simulink model "ES241A_MotAg2Meas"  (R2013b)
settings: Solver=FixedStepDiscrete  SolverMode=SingleTasking  StartTime=0.0  StopTime=1  FixedStep=0.002  RelTol=1e-3
undefined symbols (not defined in the file): ARCHGLBPRM_2PI_ULS_F32, FLTINJ_MOTAG2MEAS_MOTAG2MECL, MOTAG2ANSINCOSFLTFAILSTEP_CNT_U16, MOTAG2ANSINCOSFLTPASSSTEP_CNT_U16, MotAg2MeasOffs, MOTAG2MECLMAX_MOTREV_F32, MOTAG2MECLMIN_MOTREV_F32, NtcNr1, NtcSts1, sigbuilder_block, VALMAXERR_VOLTSQD_F32, VALMINERR_VOLTSQD_F32
libraries: simulink x12, NxtrLim x2, FloatToFixd x1, NxtrMath x1
(part 1 of 3)
settings Model: reqMgrSettings="100 S'doors','misc'{{S'surrogatepath','savemodel','savesurrogate','updateLinks','doorsLinks2sl','slLinks2Doors','purgeDoors','purgeSimulink','detaillevel','surrogateId','synctime'{{T\"./$ModelName$\",M[1],M[1],M[0],M[0],M[0],M[0],M[0],M[1],T\"\",T\"\"}},S'mode','pathStorage'{{T\"generic\",T\"modelRelative\"}}}}"  PauseTimes=0.04  Creator=KPIT  LastModifiedBy=TZBSJD
settings SolverCC: AutoInsertRateTranBlk=on  InsertRTBMode=Always
settings DataIOCC: LimitDataPoints=off  SaveFormat=Structure  ReturnWorkspaceOutputs=on
settings OptimizationCC: BlockReduction=off  InlineParams=on  ZeroExternalMemoryAtStartup=off  ZeroInternalMemoryAtStartup=off  OptimizeModelRefInitCode=on  LifeSpan=1
settings DebuggingCC: SignalInfNanChecking=error  SignalRangeChecking=warning  UnderspecifiedInitializationDetection=Simplified  SolverPrmCheckMsg=error  InheritedTsInSrcMsg=error  DiscreteInheritContinuousMsg=error  SingleTaskRateTransMsg=error  TasksWithSamePriorityMsg=error  SigSpecEnsureSampleTimeMsg=error  CheckMatrixSingularityMsg=error  ParameterUnderflowMsg=error  ParameterPrecisionLossMsg=error  ParameterTunabilityLossMsg=error  FixptConstUnderflowMsg=warning  FixptConstOverflowMsg=warning  VectorMatrixConversionMsg=error  SignalLabelMismatchMsg=error  UnconnectedInputMsg=error  UnconnectedOutputMsg=error  UnconnectedLineMsg=error  SFcnCompatibilityMsg=error  UniqueDataStoreMsg=warning  BusObjectLabelMismatch=error  RootOutportRequireBusObject=error  AssertControl=DisableAll  ModelReferenceIOMsg=error  ModelReferenceVersionMismatchMessage=warning  ModelReferenceIOMismatchMessage=error  ModelReferenceCSMismatchMessage=warning  ModelReferenceDataLoggingMessage=error  StateNameClashWarn=warning  StrictBusMsg=ErrorOnBusTreatedAsVector  NonBusSignalsTreatedAsBus=error  SFUnexpectedBacktrackingDiag=error  SFInvalidInputDataAccessInChartInitDiag=error  SFNoUnconditionalDefaultTransitionDiag=error  SFTransitionOutsideNaturalParentDiag=error  SFUnconditionalTransitionShadowingDiag=error  SFUndirectedBroadcastEventsDiag=error
settings ModelReferenceCC: ModelReferenceNumInstancesAllowed=Single
settings SFSimCC: SimGenImportedTypeDefs=on
settings RTWCC: SystemTargetFile=autosar.tlc  GenCodeOnly=on  TemplateMakefile=ert_default_tmf  Description=AUTOSAR  GenerateReport=on  ProcessScript=autosar_make_rtw_hook  LaunchReport=on
settings CodeAppCC: GenerateComments=off  IgnoreCustomStorageClasses=off  CustomSymbolStrType=$N$R$M  CustomSymbolStrBlkIO=$N$M  SimulinkBlockComments=off
settings STFCustomTargetCC: ParMdlRefBuildCompliant=on  CompOptLevelCompliant=on  IncludeMdlTerminateFcn=off  CombineOutputUpdateFcns=on  SuppressErrorStatus=on  ERTFirstTimeCompliant=on  ERTCustomFileBanners=on  SupportNonFinite=off  SupportComplex=off  SupportContinuousTime=off  SupportNonInlinedSFcns=off  MATLABClassNameForMDSCustomization=Simulink.SoftwareTarget.ERTCustomization  AutosarCompliant=on  GRTInterface=off  SystemTargetFile=autosar.tlc
settings ERTTargetCC: CodeReplacementLibrary=ANSI_C  ConcurrentExecutionCompliant=off  IncludeMdlTerminateFcn=off  SuppressErrorStatus=on  SupportNonFinite=off  SupportComplex=off  ModelStepFunctionPrototypeControlCompliant=off  CPPClassGenCompliant=off  AutosarCompliant=on  InlinedParameterPlacement=NonHierarchical  ERTCustomFileTemplate=example_file_process.tlc  EnableUserReplacementTypes=on

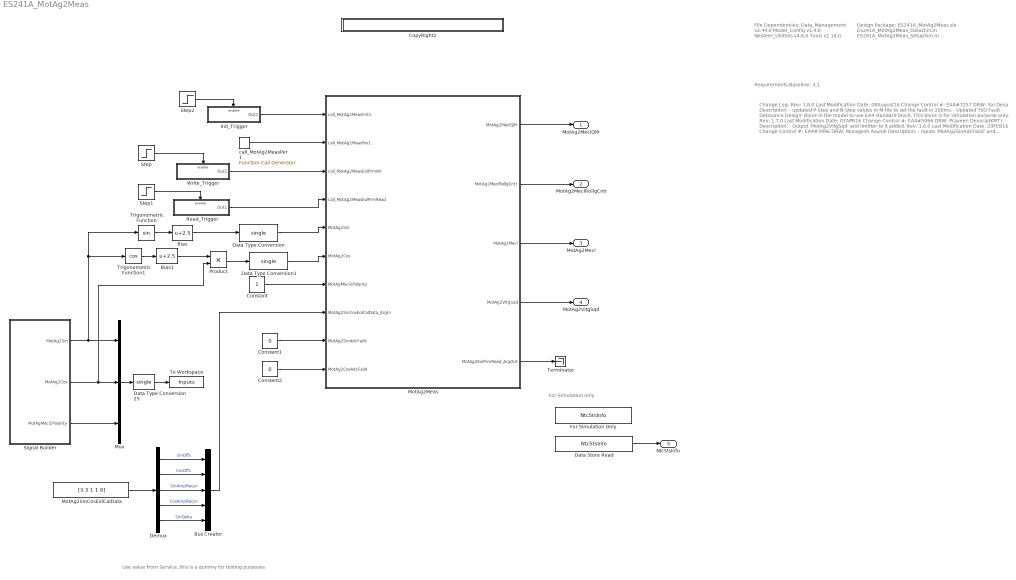
== system ES241A_MotAg2Meas ==
  note: Requirements Baseline: 3.1
  note: File Dependencies:
      |
      | Data_Management v2.44.0
      | Model_Config v1.4.0
      | Nexteer_Utilities v4.6.0
      | Tools v1.14.0
  note: Change Log:
      | Rev: 1.8.0
      | Last Modification Date: 08August16
      | Change Control #: EA4#7257
      | DRW: Sai Desu
      | Description:
      |      - updated P-Step and N-Step values in M-file to set the fault in 200ms.
      |      - Updated 'ISO Fault Debounce Design' Block in the model to use EA4 standard block.
      |        This block is for simulation purpose only.
      |
      | Rev: 1.7.0
      | Last Modification Date: 07APR16
      | Change Control #: EA4#5066
      | DRW: Praveen Devaraj(KPIT)
      | Description:
      |      - Output 'MotAg2VltgSqd' and limitter to it added.
      |
      | Rev: 1.6.0
      | Last Modification Date: 29FEB16
      | Change Control #: EA4#3996
      | DRW: Muragesh Asundi
      | Description:
      |      - Inputs 'MotAg2SinAdcFaild' and 'MotAg2CosAdcFaild' and logic related
      |        to these inputs added
      |
      | Rev: 1.5.0
      | Last Modification Date: 16DEC15
      | Change Control #: EA4#2797
      | DRW: Keyurkumar Gondaliya/Muragesh Asundi
      | Description:
      |      - Input 'MtrAg2SinCosEolCalDataCrc_ArgIn' and output 'MotAg2SinCosWrResp_ArgOut' removed
      |      - 'MtrAg2EolPrmReadCrc_ArgOut' and logic related to it removed. DD updated.
      |      - Fixed anlomaly CR EA4#2565
      |
      | Rev: 1.4.0
      | Last Modification Date: 18NOV15
      | Change Control #: EA4#2526
      | DRW: Erlenbeck
      | Description:
      | 	Change the output type of MotAg2Mecl from f32 to u0p16
      |
      | Rev: 1.3.0
      | Last Modification Date: 10.26.2015
      | Change Control #: EA4#1460
      | DRW: Muragesh Asundi
      | Description:
      | - Remove Mod block
      | - Change CRC length from 10 to 20
      | - Naming conventions for Nstep & Pstep changed as PASS and Fail step
      | - Add limitter for output 'MotAg2Mecl'
      |
      | Rev: 1.2.0
      | Last Modification Date: 08.27.2015
      | Change Control #: EA4#1421
      | DRW: Muragesh Asundi
      | Description:
      | - Changed I/O from the service functions from an array of f32 to the EOL parameter struct
      | - Removed 2 from the struct
      | - Changed IO signals names from MtrPos to MotAg
      | - PIM MotAg2MeclRollgCntrPrev added
      |
      | Rev: 1.1.0
      | Last Modification Date: 08.24.2015
      | Change Control #: EA4#1356
      | DRW: Muragesh Asundi
      | Description:
      | - Added Fault Injection block for output MotAg2Mecl
      |
      | v1.0.0
      | Date: 18-Aug-2015
      | Change Control #: EA4#1007
      | DRW:  Aditya Tikekar
      | Description:
      | - Initial Release of EA3 1.0.0
  note: Design Package:
      |
      | ES241A_MotAg2Meas.slx
      | ES241A_MotAg2Meas_DataDict.m
      | ES241A_MotAg2Meas_SetupSim.m
  note: Use value from Service, this is a dummy for testing purposes
  note: For Simulation only
  Bias : Bias  Bias=2.5
  Bias1 : Bias  Bias=2.5
  Bus Creator : BusCreator  Inputs='SinOffs','CosOffs','SinAmpRecpr','CosAmpRecpr','SinDelta'  OutDataTypeStr=Bus: MotAgMeasEolPrmRec1  NonVirtualBus=on
  Constant : Constant
  Constant1 : Constant  Value=0  OutDataTypeStr=boolean
  Constant2 : Constant  Value=0  OutDataTypeStr=boolean
  CopyRight2 : Subsystem  Description=|  mask(Copyright Information){none=on}
      | Copyright info block.                                               
      |                                                                     
      | Place copyright information at the top of every subsystem in design.
      mask prompts: none "No parameters"
      mask help: Place copyright information at the top of every subsystem in design.
      mask Display:
      | NxtrConf = 'Nexteer Confidential';
      | 
      | sys = bdroot; %handle for the current model ("system")
      | first = get_param(sys,'Created');
      | if(isempty(first))
      |     first = datestr(now,'yyyy');
      | else
      |     first = first(end-3:end);  %year is last four digits
      | end
      | 
      | last = get_param(sys,'LastModifiedDate');
      | if isempty(last)
      |     last = datestr(now,'yyyy');
      | else
      |     last = last(end-3:end);
      | end
      | 
      | if strcmp(first,last)
      |     fprintf('%s -- Copyright %s Nexteer',NxtrConf,first)
      | else
      |     fprintf('%s -- %s%s- %s Nexteer',NxtrConf,char(169),first,last)
      | end
  Data Store Read : DataStoreRead  DataStoreName=NtcStsInfo  SampleTime=0.002
  Data Type Conversion : DataTypeConversion  OutDataTypeStr=single
  Data Type Conversion1 : DataTypeConversion  OutDataTypeStr=single
  Data Type Conversion25 : DataTypeConversion  OutDataTypeStr=single
  Demux : Demux  Outputs=5
  For Simulation Only : DataStoreMemory  DataStoreName=NtcStsInfo  ReadBeforeWriteMsg=warning  WriteAfterWriteMsg=warning  WriteAfterReadMsg=warning
  Init_Trigger : Subsystem  TreatAsAtomicUnit=on
  MotAg2Meas : Subsystem
  MotAg2SinCosEolCalData : Constant  Value=[3 3 1 1 0]  OutDataTypeStr=single
  Mux : Mux  Inputs=3
  Product : Product
  Read_Trigger : Subsystem  TreatAsAtomicUnit=on
  Signal Builder : Subsystem  Tag=STV Subsys  LoadFcn=sigbuilder_block('load');  StartFcn=sigbuilder_block('start');  StopFcn=sigbuilder_block('stop');  ClipboardFcn=sigbuilder_block('clipboard');  mask(Sigbuilder block){}
      mask help: Simulink:masks:SigbuilderBlock_MD
      mask init:
      | if ~strcmp(get_param(bdroot(gcbh),'SimulationStatus'),'stopped') tuvar = sigbuilder_block('maskInit'); end
      settings: CopyFcn=sigbuilder_block('copy');  DeleteFcn=sigbuilder_block('delete');  ModelCloseFcn=sigbuilder_block('modelClose');  PreSaveFcn=sigbuilder_block('preSave');  PauseFcn=sigbuilder_block('pause');  ContinueFcn=sigbuilder_block('continue');  NameChangeFcn=sigbuilder_block('namechange');  OpenFcn=sigbuilder_block('open',[-1024.5 0 1024.5 519 ]);  CloseFcn=sigbuilder_block('close');
      mask Display: plot(0, 0, 100, 100,[2, 2, 32, 32, 2], [68, 8, 8, 68, 68],[32, 2], [38, 38], [32, 19, 2],[53, 60, 44], [32, 17, 17, 2],[16, 16, 31, 31]);txt = getActiveGroup(gcbh);text(2, 100, txt,'verticalAlignment', 'top');
  Step : Step  Time=0.25  SampleTime=0
  Step1 : Step  Time=0.006  SampleTime=0
  Step2 : Step  Time=0.002  Before=1  After=0  SampleTime=0
  Terminator : Terminator
  To Workspace : ToWorkspace  VariableName=Inputs  SampleTime=-1
  Trigonometric Function : Trigonometry
  Trigonometric Function1 : Trigonometry  Operator=cos
  Write_Trigger : Subsystem  TreatAsAtomicUnit=on
  call_MotAg2MeasPer1 : simulink/Ports & Subsystems/Function-Call Generator  RequirementInfo={} %GIDa_bc46352c_0424_4e0d_b48f_57630b448788  sample_time=0.002  numberOfIterations=1
  MotAg2MeclQlfr : Outport  RequirementInfo={} %GIDa_13339e60_d901_415b_99de_5a5f823e821e
  MotAg2MeclRollgCntr : Outport  RequirementInfo={} %GIDa_64b1d497_6b46_497b_9639_71fa2240e4cb  Port=2
  MotAg2Mecl : Outport  RequirementInfo={} %GIDa_77db205e_a8cc_41ed_9223_bd045923b052  Port=3
  MotAg2VltgSqd : Outport  Port=4
  NtcStsInfo : Outport  RequirementInfo={} %GIDa_305790cc_b4da_485d_acf3_4b5d9228ea47  Port=5
  wires:
  call_MotAg2MeasPer1/1 -> MotAg2Meas/2(call_MotAg2MeasPer1)
  MotAg2Meas/5(MotAg2EolPrmRead_ArgOut) -> Terminator/1
  Mux/1 -> Data Type Conversion25/1
  Data Type Conversion25/1 -> To Workspace/1
  Constant/1 -> MotAg2Meas/7(MotAgMecl2Polarity)
  Bias/1 -> Data Type Conversion/1
  Step/1 -> Write_Trigger/Enable
  Step1/1 -> Read_Trigger/Enable
  Write_Trigger/1(Out1) -> MotAg2Meas/3(call_MotAg2MeasEolPrmWr)
  Read_Trigger/1(Out1) -> MotAg2Meas/4(call_MotAg2MeasEolPrmRead)
  Step2/1 -> Init_Trigger/Enable
  Init_Trigger/1(Out1) -> MotAg2Meas/1(call_MotAg2MeasInit1)
  Signal Builder/1(MotAg2Sin) -> Mux/1, Trigonometric Function/1, Trigonometric Function1/1
  Signal Builder/3(MotAgMecl2Polarity) -> Mux/3
  Signal Builder/2(MotAg2Cos) -> Product/2, Mux/2
  MotAg2Meas/1(MotAg2MeclQlfr) -> MotAg2MeclQlfr/1
  MotAg2Meas/2(MotAg2MeclRollgCntr) -> MotAg2MeclRollgCntr/1
  MotAg2Meas/3(MotAg2Mecl) -> MotAg2Mecl/1
  Trigonometric Function/1 -> Bias/1
  Trigonometric Function1/1 -> Bias1/1
  Bias1/1 -> Product/1
  Data Type Conversion/1 -> MotAg2Meas/5(MotAg2Sin)
  Data Type Conversion1/1 -> MotAg2Meas/6(MotAg2Cos)
  Product/1 -> Data Type Conversion1/1
  Demux/5 -> Bus Creator/5  "SinDelta"
  Demux/4 -> Bus Creator/4  "CosAmpRecpr"
  Demux/2 -> Bus Creator/2  "CosOffs"
  Demux/3 -> Bus Creator/3  "SinAmpRecpr"
  Demux/1 -> Bus Creator/1  "SinOffs"
  MotAg2SinCosEolCalData/1 -> Demux/1
  Bus Creator/1 -> MotAg2Meas/8(MotAg2SinCosEolCalData_ArgIn)
  Constant2/1 -> MotAg2Meas/10(MotAg2CosAdcFaild)
  Constant1/1 -> MotAg2Meas/9(MotAg2SinAdcFaild)
  Data Store Read/1 -> NtcStsInfo/1
  MotAg2Meas/4(MotAg2VltgSqd) -> MotAg2VltgSqd/1

== system ES241A_MotAg2Meas/CopyRight2 ==

== system ES241A_MotAg2Meas/Init_Trigger ==
  Enable : EnablePort
  Function-Call Generator1 : simulink/Ports & Subsystems/Function-Call Generator  sample_time=0  numberOfIterations=1
  Out1 : Outport
  wires:
  Function-Call Generator1/1 -> Out1/1

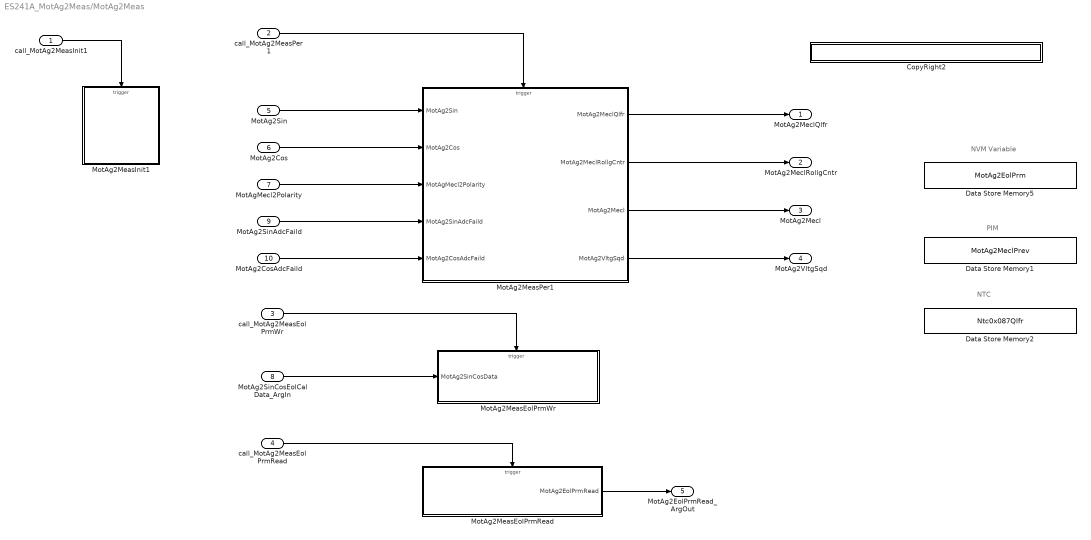
== system ES241A_MotAg2Meas/MotAg2Meas ==
  note: PIM
  note: NTC
  note: NVM Variable
  call_MotAg2MeasInit1 : Inport
  call_MotAg2MeasPer1 : Inport  Port=2
  call_MotAg2MeasEolPrmWr : Inport  Port=3
  call_MotAg2MeasEolPrmRead : Inport  Port=4
  MotAg2Sin : Inport  RequirementInfo={'linktype_rmi_doors' '0000cf65 (/E-STEER Core/SubSystem Specifications/Electrical Actuator/Control Module/FDD Module Requirements/EA4/ES241A_MotAg2Meas)' '#ES241A_49' 'true' 'REQ: ES241A_49' '' } %GIDa_7d298e34_c05b_439c_ad49_94e8d3b397f3  Port=5
  MotAg2Cos : Inport  RequirementInfo={'linktype_rmi_doors' '0000cf65 (/E-STEER Core/SubSystem Specifications/Electrical Actuator/Control Module/FDD Module Requirements/EA4/ES241A_MotAg2Meas)' '#ES241A_48' 'true' 'REQ: ES241A_48' '' } %GIDa_73391b37_a5e9_4145_aca0_ac09474f9974  Port=6
  MotAgMecl2Polarity : Inport  RequirementInfo={'linktype_rmi_doors' '0000cf65 (/E-STEER Core/SubSystem Specifications/Electrical Actuator/Control Module/FDD Module Requirements/EA4/ES241A_MotAg2Meas)' '#ES241A_65' 'true' 'REQ: ES241A_65' '' } %GIDa_856eeb3a_bbb6_4880_ab78_80a15c90fc09  Port=7
  MotAg2SinCosEolCalData_ArgIn : Inport  Port=8  OutDataTypeStr=Bus: MotAgMeasEolPrmRec1
  MotAg2SinAdcFaild : Inport  RequirementInfo={'linktype_rmi_doors' '0000cf65 (/E-STEER Core/SubSystem Specifications/Electrical Actuator/Control Module/FDD Module Requirements/EA4/ES241A_MotAg2Meas)' '#ES241A_146' 'true' 'REQ: ES241A_146' '' } %GIDa_82f7f128_b8c8_49c8_b664_98de2aa09858  Port=9
  MotAg2CosAdcFaild : Inport  RequirementInfo={'linktype_rmi_doors' '0000cf65 (/E-STEER Core/SubSystem Specifications/Electrical Actuator/Control Module/FDD Module Requirements/EA4/ES241A_MotAg2Meas)' '#ES241A_145' 'true' 'REQ: ES241A_145' '' } %GIDa_a44d5a9e_6b3c_447d_b1ad_61e623b783fe  Port=10
  CopyRight2 : Subsystem  Description=|  mask(Copyright Information){none=on}
      | Copyright info block.                                               
      |                                                                     
      | Place copyright information at the top of every subsystem in design.
      mask prompts: none "No parameters"
      mask help: Place copyright information at the top of every subsystem in design.
      mask Display:
      | NxtrConf = 'Nexteer Confidential';
      | 
      | sys = bdroot; %handle for the current model ("system")
      | first = get_param(sys,'Created');
      | if(isempty(first))
      |     first = datestr(now,'yyyy');
      | else
      |     first = first(end-3:end);  %year is last four digits
      | end
      | 
      | last = get_param(sys,'LastModifiedDate');
      | if isempty(last)
      |     last = datestr(now,'yyyy');
      | else
      |     last = last(end-3:end);
      | end
      | 
      | if strcmp(first,last)
      |     fprintf('%s -- Copyright %s Nexteer',NxtrConf,first)
      | else
      |     fprintf('%s -- %s%s- %s Nexteer',NxtrConf,char(169),first,last)
      | end
  Data Store Memory1 : DataStoreMemory  DataStoreName=MotAg2MeclPrev  StateMustResolveToSignalObject=on
  Data Store Memory2 : DataStoreMemory  DataStoreName=Ntc0x087Qlfr
  Data Store Memory5 : DataStoreMemory  DataStoreName=MotAg2EolPrm  InitialValue=[]  OutDataTypeStr=Bus: MotAgMeasEolPrmRec1  StateMustResolveToSignalObject=on
  MotAg2MeasEolPrmRead : Subsystem  RequirementInfo={'linktype_rmi_doors' '0000cf65 (/E-STEER Core/SubSystem Specifications/Electrical Actuator/Control Module/FDD Module Requirements/EA4/ES241A_MotAg2Meas)' '#ES241A_135' 'true' 'REQ: ES241A_135' '' } %GIDa_cb0be6f7_2f31_479b_8294_40ee3e4aca08  TreatAsAtomicUnit=on
  MotAg2MeasEolPrmWr : Subsystem  RequirementInfo={'linktype_rmi_doors' '0000cf65 (/E-STEER Core/SubSystem Specifications/Electrical Actuator/Control Module/FDD Module Requirements/EA4/ES241A_MotAg2Meas)' '#ES241A_32' 'true' 'REQ: ES241A_32' '' } %GIDa_9fac367d_a0e4_41dd_ba23_6b4ec78d47c5
  MotAg2MeasInit1 : Subsystem  TreatAsAtomicUnit=on
  MotAg2MeasPer1 : Subsystem  ClipboardFcn=Priority=%<Priority>  TreatAsAtomicUnit=on
  MotAg2MeclQlfr : Outport  RequirementInfo={'linktype_rmi_doors' '0000cf65 (/E-STEER Core/SubSystem Specifications/Electrical Actuator/Control Module/FDD Module Requirements/EA4/ES241A_MotAg2Meas)' '#ES241A_113' 'true' 'REQ: ES241A_113' '' } %GIDa_ad4892e3_f342_4a8c_9fb3_dbca1d6629f8
  MotAg2MeclRollgCntr : Outport  RequirementInfo={'linktype_rmi_doors' '0000cf65 (/E-STEER Core/SubSystem Specifications/Electrical Actuator/Control Module/FDD Module Requirements/EA4/ES241A_MotAg2Meas)' '#ES241A_114' 'true' 'REQ: ES241A_114' '' } %GIDa_5e51ab32_dc6c_4788_a108_d1ac524f47aa  Port=2
  MotAg2Mecl : Outport  RequirementInfo={'linktype_rmi_doors' '0000cf65 (/E-STEER Core/SubSystem Specifications/Electrical Actuator/Control Module/FDD Module Requirements/EA4/ES241A_MotAg2Meas)' '#ES241A_51' 'true' 'REQ: ES241A_51' '' } %GIDa_b54aa487_7774_4247_9155_2f93ac20eae7  Port=3
  MotAg2VltgSqd : Outport  RequirementInfo={'linktype_rmi_doors' '0000cf65 (/E-STEER Core/SubSystem Specifications/Electrical Actuator/Control Module/FDD Module Requirements/EA4/ES241A_MotAg2Meas)' '#ES241A_151' 'true' 'REQ: ES241A_151' '' } %GIDa_822906ad_a1cb_4535_b465_c74a6fe6a8d1  Port=4
  MotAg2EolPrmRead_ArgOut : Outport  Port=5  OutDataTypeStr=Bus: MotAgMeasEolPrmRec1
  wires:
  call_MotAg2MeasPer1/1 -> MotAg2MeasPer1/Trigger
  MotAg2Sin/1 -> MotAg2MeasPer1/1(MotAg2Sin)
  MotAgMecl2Polarity/1 -> MotAg2MeasPer1/3(MotAgMecl2Polarity)
  MotAg2Cos/1 -> MotAg2MeasPer1/2(MotAg2Cos)
  MotAg2MeasPer1/1(MotAg2MeclQlfr) -> MotAg2MeclQlfr/1
  MotAg2MeasPer1/2(MotAg2MeclRollgCntr) -> MotAg2MeclRollgCntr/1
  MotAg2MeasPer1/3(MotAg2Mecl) -> MotAg2Mecl/1
  call_MotAg2MeasInit1/1 -> MotAg2MeasInit1/Trigger
  call_MotAg2MeasEolPrmWr/1 -> MotAg2MeasEolPrmWr/Trigger
  MotAg2MeasEolPrmRead/1(MotAg2EolPrmRead) -> MotAg2EolPrmRead_ArgOut/1
  call_MotAg2MeasEolPrmRead/1 -> MotAg2MeasEolPrmRead/Trigger
  MotAg2SinCosEolCalData_ArgIn/1 -> MotAg2MeasEolPrmWr/1(MotAg2SinCosData)
  MotAg2SinAdcFaild/1 -> MotAg2MeasPer1/4(MotAg2SinAdcFaild)
  MotAg2CosAdcFaild/1 -> MotAg2MeasPer1/5(MotAg2CosAdcFaild)
  MotAg2MeasPer1/4(MotAg2VltgSqd) -> MotAg2VltgSqd/1

== system ES241A_MotAg2Meas/Read_Trigger ==
  Enable : EnablePort
  Function-Call Generator1 : simulink/Ports & Subsystems/Function-Call Generator  sample_time=0.002  numberOfIterations=1
  Out1 : Outport
  wires:
  Function-Call Generator1/1 -> Out1/1

== system ES241A_MotAg2Meas/Signal Builder ==
  Demux : Demux  Tag=STV Demux  Outputs=3
  FromWs : FromWorkspace  Tag=STV FromWs  VariableName=tuvar  SampleTime=0
      SigBuilderData=|
      | common.afterFinalStr = 'Extrapolate'
      | common.sampleTime = 0
      | dataSet(1).timeRange = [0 1]
      | dataSet(1).name = 'MotAg2CosCmp_Calc'
      | dataSet(2).timeRange = [0 1]
      | dataSet(2).name = 'MotAg2SinCmp_Calc'
      | dataSet(3).timeRange = [0 0.04]
      | dataSet(3).name = 'CosTheta_Calc'
      | dataSet(4).timeRange = [0 0.04]
      | dataSet(4).name = 'MotAg2Mecl_Calc_Polarity_1'
      | dataSet(5).timeRange = [0 0.04]
      | dataSet(5).name = 'MotAg2Mecl_Calc_Polarity_-1'
      | dataSet(6).timeRange = [0 0.25]
      | dataSet(6).name = 'ISO_Fault'
      | dataSet(7).timeRange = [0 1]
      | dataSet(7).name = 'RollCntr>255'
      | dataSet(8).timeRange = [0 1]
      | dataSet(8).name = 'NoFault'
      | sbobj.Name = 'Signal Builder'
      | sbobj.Groups(1).Name = 'MotAg2CosCmp_Calc'
      | sbobj.Groups(1).Signals(1).Name = 'MotAg2Sin'
      | sbobj.Groups(1).Signals(1).XData = [0 0.002 0.004 0.006 0.008 0.01 0.012 0.014 0.016 0.018 0.02 0.02 0.022 0.022 0.024 0.026 0.028 0.03 0.032 0.034 0.036 0.038 0.04 0.04 1]
      | sbobj.Groups(1).Signals(1).YData = [0 2.5 4.5 5 4.5 2.5 0 2.5 4.5 5 4.5 4.45 2.3 2.5 0 2.5 4.5 5 4.5 2.5 0 2.5 4.5 1.95 1.95]
      | sbobj.Groups(1).Signals(2).Name = 'MotAg2Cos'
      | sbobj.Groups(1).Signals(2).XData = [0 0.002 0.004 0.006 0.008 0.01 0.012 0.014 0.016 0.018 0.02 0.022 0.024 0.026 0.028 0.03 0.032 0.034 0.036 0.038 0.04 1]
      | sbobj.Groups(1).Signals(2).YData = [5 4.5 2.5 0 2.5 4.5 5 4.5 2.5 0 2.5 4.5 5 4.5 2.5 0 2.5 4.5 5 4.5 2.5 2.5]
      | sbobj.Groups(1).Signals(3).Name = 'MotAgMecl2Polarity'
      | sbobj.Groups(1).Signals(3).XData = [0 0.002 0.004 0.006 0.008 0.01 0.012 0.014 0.016 0.018 0.02 0.022 0.024 0.026 0.028 0.03 0.032 0.034 0.036 0.038 0.04 1]
      | sbobj.Groups(1).Signals(3).YData = [-1 1 -1 1 -1 1 -1 0 0 0 1 -1 1 0 -1 1 -1 1 0 0 1 1]
      | sbobj.Groups(1).TimeRange = [0 1]
      | sbobj.Groups(2).Name = 'MotAg2SinCmp_Calc'
      | sbobj.Groups(2).Signals(1).Name = 'MotAg2Sin'
      | sbobj.Groups(2).Signals(1).XData = [0 0.5 0.5 1]
      | sbobj.Groups(2).Signals(1).YData = [0 6.28318 0 6.28318]
      | sbobj.Groups(2).Signals(2).Name = 'MotAg2Cos'
      | sbobj.Groups(2).Signals(2).XData = [0 0.5 0.5 1]
      | sbobj.Groups(2).Signals(2).YData = [1 1 0 0]
      | sbobj.Groups(2).Signals(3).Name = 'MotAgMecl2Polarity'
      | sbobj.Groups(2).Signals(3).XData = [0 0.002 0.004 0.006 0.008 0.01 0.012 0.014 0.016 0.018 0.02 0.022 0.024 0.026 0.028 0.03 0.032 0.034 0.036 0.038 0.04 1]
      | sbobj.Groups(2).Signals(3).YData = [-1 1 -1 1 -1 1 -1 0 0 0 1 -1 1 0 -1 1 -1 1 0 0 1 1]
      | sbobj.Groups(2).TimeRange = [0 1]
      | sbobj.Groups(3).Name = 'CosTheta_Calc'
      | sbobj.Groups(3).Signals(1).Name = 'MotAg2Sin'
      | sbobj.Groups(3).Signals(1).XData = [0 0.002 0.004 0.006 0.008 0.01 0.012 0.014 0.016 0.018 0.02 0.022 0.024 0.026 0.028 0.03 0.032 0.034 0.036 0.038 0.04]
      | sbobj.Groups(3).Signals(1).YData = [0 2.5 4.5 5 4.5 2.5 0 2.5 4.5 5 4.5 2.5 0 2.5 4.5 5 4.5 2.5 0 2.5 4.5]
      | sbobj.Groups(3).Signals(2).Name = 'MotAg2Cos'
      | sbobj.Groups(3).Signals(2).XData = [0 0.002 0.004 0.006 0.008 0.01 0.012 0.014 0.016 0.018 0.02 0.022 0.024 0.026 0.028 0.03 0.032 0.034 0.036 0.038 0.04]
      | sbobj.Groups(3).Signals(2).YData = [5 4.5 2.5 0 2.5 4.5 5 4.5 2.5 0 2.5 4.5 5 4.5 2.5 0 2.5 4.5 5 4.5 2.5]
      | sbobj.Groups(3).Signals(3).Name = 'MotAgMecl2Polarity'
      | sbobj.Groups(3).Signals(3).XData = [0 0.002 0.004 0.006 0.008 0.01 0.012 0.014 0.016 0.018 0.02 0.022 0.024 0.026 0.028 0.03 0.032 0.034 0.036 0.038 0.04]
      | sbobj.Groups(3).Signals(3).YData = [-1 1 -1 1 -1 1 -1 0 0 0 1 -1 1 0 -1 1 -1 1 0 0 1]
      | sbobj.Groups(3).TimeRange = [0 0.04]
      | sbobj.Groups(4).Name = 'MotAg2Mecl_Calc_Polarity_1'
      | sbobj.Groups(4).Signals(1).Name = 'MotAg2Sin'
      | sbobj.Groups(4).Signals(1).XData = [0 0.002 0.004 0.006 0.008 0.01 0.012 0.014 0.016 0.018 0.02 0.022 0.024 0.026 0.028 0.03 0.032 0.034 0.036 0.038 0.04]
      | sbobj.Groups(4).Signals(1).YData = [0 2.5 4.5 5 4.5 2.5 0 2.5 4.5 5 4.5 2.5 0 2.5 4.5 5 4.5 2.5 0 2.5 4.5]
      | sbobj.Groups(4).Signals(2).Name = 'MotAg2Cos'
      | sbobj.Groups(4).Signals(2).XData = [0 0.002 0.004 0.006 0.008 0.01 0.012 0.014 0.016 0.018 0.02 0.022 0.024 0.026 0.028 0.03 0.032 0.034 0.036 0.038 0.04]
      | sbobj.Groups(4).Signals(2).YData = [5 4.5 2.5 0 2.5 4.5 5 4.5 2.5 0 2.5 4.5 5 4.5 2.5 0 2.5 4.5 5 4.5 2.5]
      | sbobj.Groups(4).Signals(3).Name = 'MotAgMecl2Polarity'
      | sbobj.Groups(4).Signals(3).XData = [0 0.002 0.004 0.006 0.008 0.01 0.012 0.014 0.016 0.018 0.02 0.022 0.024 0.026 0.028 0.03 0.032 0.034 0.036 0.038 0.04]
      | sbobj.Groups(4).Signals(3).YData = [1 1 1 1 1 1 1 1 1 1 1 1 1 1 1 1 1 1 1 1 1]
      | sbobj.Groups(4).TimeRange = [0 0.04]
      | sbobj.Groups(5).Name = 'MotAg2Mecl_Calc_Polarity_-1'
      | sbobj.Groups(5).Signals(1).Name = 'MotAg2Sin'
      | sbobj.Groups(5).Signals(1).XData = [0 0.002 0.004 0.006 0.008 0.01 0.012 0.014 0.016 0.018 0.02 0.022 0.024 0.026 0.028 0.03 0.032 0.034 0.036 0.038 0.04]
      | sbobj.Groups(5).Signals(1).YData = [0 2.5 4.5 5 4.5 2.5 0 2.5 4.5 5 4.5 2.5 0 2.5 4.5 5 4.5 2.5 0 2.5 4.5]
      | sbobj.Groups(5).Signals(2).Name = 'MotAg2Cos'
      | sbobj.Groups(5).Signals(2).XData = [0 0.002 0.004 0.006 0.008 0.01 0.012 0.014 0.016 0.018 0.02 0.022 0.024 0.026 0.028 0.03 0.032 0.034 0.036 0.038 0.04]
      | sbobj.Groups(5).Signals(2).YData = [5 4.5 2.5 0 2.5 4.5 5 4.5 2.5 0 2.5 4.5 5 4.5 2.5 0 2.5 4.5 5 4.5 2.5]
      | sbobj.Groups(5).Signals(3).Name = 'MotAgMecl2Polarity'
      | sbobj.Groups(5).Signals(3).XData = [0 0.002 0.004 0.006 0.008 0.01 0.012 0.014 0.016 0.018 0.02 0.022 0.024 0.026 0.028 0.03 0.032 0.034 0.036 0.038 0.04]
      | sbobj.Groups(5).Signals(3).YData = [-1 -1 -1 -1 -1 -1 -1 -1 -1 -1 -1 -1 -1 -1 -1 -1 -1 -1 -1 -1 -1]
      | sbobj.Groups(5).TimeRange = [0 0.04]
      | sbobj.Groups(6).Name = 'ISO_Fault'
      | sbobj.Groups(6).Signals(1).Name = 'MotAg2Sin'
      | sbobj.Groups(6).Signals(1).XData = [0 0.002 0.004 0.006 0.008 0.01 0.012 0.014 0.016 0.018 0.02 0.022 0.024 0.026 0.028 0.03 0.032 0.034 0.036 0.038 0.04 0.042 0.044 0.046 0.048 0.05 0.052 0.054 0.056 0.058 0.06 0.062 0.064 0.066 0.068 0.07 0.072 0.074 0.076 0.078 0.08 0.082 0.084 0.086 0.088 0.09 0.092 0.094 0.096 0.098 0.1 0.102 0.104 0.106 0.108 0.11 0.112 0.114 0.116 0.118 0.12 0.122 0.124 0.126 0.128 0.13 0.132 0.134 0.136 0.138 0.14 0.142 0.144 0.146 0.148 0.15 0.152 0.154 0.156 0.158 0.16 0.162 0.164 0.166 0.168 0.17 0.172 0.174 0.176 0.178 0.18 0.182 0.184 0.186 0.188 0.19 0.192 0.194 0.196 0.198 0.2 0.202 0.204 0.206 0.208 0.21 0.212 0.214 0.216 0.218 0.22 0.222 0.224 0.226 0.228 0.23 0.232 0.234 0.236 0.238 0.24 0.242 0.244 0.246 0.248 0.25]
      | sbobj.Groups(6).Signals(1).YData = [0 2.5 4.5 5 4.5 2.5 0 2.5 4.5 5 4.5 2.5 0 2.5 4.5 5 4.5 2.5 0 2.5 4.5 5 4.5 2.5 0 2.5 4.5 5 4.5 2.5 0 2.5 4.5 5 4.5 2.5 0 2.5 4.5 5 4.5 2.5 0 2.5 4.5 5 4.5 2.5 0 2.5 4.5 5 4.5 2.5 0 2.5 4.5 5 4.5 2.5 0 2.5 4.5 5 4.5 2.5 0 2.5 4.5 5 4.5 2.5 0 2.5 4.5 5 4.5 2.5 0 2.5 4.5 5 4.5 2.5 0 2.5 4.5 5 4.5 2.5 0 2.5 4.5 5 4.5 2.5 0 2.5 4.5 5 4.5 2.5 0 2.5 4.5 5 4.5 2.5 0 2.5 4.5 5 4.5 2.5 0 2.5 4.5 5 4.5 2.5 0 2.5 4.5 5 4.5 2.5]
      | sbobj.Groups(6).Signals(2).Name = 'MotAg2Cos'
      | sbobj.Groups(6).Signals(2).XData = [0 0.002 0.004 0.006 0.008 0.01 0.012 0.014 0.016 0.018 0.02 0.022 0.024 0.026 0.028 0.03 0.032 0.034 0.036 0.038 0.04 0.042 0.044 0.046 0.048 0.05 0.052 0.054 0.056 0.058 0.06 0.062 0.064 0.066 0.068 0.07 0.072 0.074 0.076 0.078 0.08 0.082 0.084 0.086 0.088 0.09 0.092 0.094 0.096 0.098 0.1 0.102 0.104 0.106 0.108 0.11 0.112 0.114 0.116 0.118 0.12 0.122 0.124 0.126 0.128 0.13 0.132 0.134 0.136 0.138 0.14 0.142 0.144 0.146 0.148 0.15 0.152 0.154 0.156 0.158 0.16 0.162 0.164 0.166 0.168 0.17 0.172 0.174 0.176 0.178 0.18 0.182 0.184 0.186 0.188 0.19 0.192 0.194 0.196 0.198 0.2 0.202 0.204 0.206 0.208 0.21 0.212 0.214 0.216 0.218 0.22 0.222 0.224 0.226 0.228 0.23 0.232 0.234 0.236 0.238 0.24 0.242 0.244 0.246 0.248 0.25]
      | sbobj.Groups(6).Signals(2).YData = [5 4.5 2.5 0 2.5 4.5 5 4.5 2.5 0 2.5 4.5 5 4.5 2.5 0 2.5 4.5 5 4.5 2.5 0 2.5 4.5 5 4.5 2.5 0 2.5 4.5 5 4.5 2.5 0 2.5 4.5 5 4.5 2.5 0 2.5 4.5 5 4.5 2.5 0 2.5 4.5 5 4.5 2.5 0 2.5 4.5 5 4.5 2.5 0 2.5 4.5 5 4.5 2.5 0 2.5 4.5 5 4.5 2.5 0 2.5 4.5 5 4.5 2.5 0 2.5 4.5 5 4.5 2.5 0 2.5 4.5 5 4.5 2.5 0 2.5 4.5 5 4.5 2.5 0 2.5 4.5 5 4.5 2.5 0 2.5 4.5 5 4.5 2.5 0 2.5 4.5 5 4.5 2.5 0 2.5 4.5 5 4.5 2.5 0 2.5 4.5 5 4.5 2.5 0 2.5 4.5]
      | sbobj.Groups(6).Signals(3).Name = 'MotAgMecl2Polarity'
      | sbobj.Groups(6).Signals(3).XData = [0 0.002 0.004 0.006 0.008 0.01 0.012 0.014 0.016 0.018 0.02 0.022 0.024 0.026 0.028 0.03 0.032 0.034 0.036 0.038 0.04 0.042 0.044 0.046 0.048 0.05 0.052 0.054 0.056 0.058 0.06 0.062 0.064 0.066 0.068 0.07 0.072 0.074 0.076 0.078 0.08 0.082 0.084 0.086 0.088 0.09 0.092 0.094 0.096 0.098 0.1 0.102 0.104 0.106 0.108 0.11 0.112 0.114 0.116 0.118 0.12 0.122 0.124 0.126 0.128 0.13 0.132 0.134 0.136 0.138 0.14 0.142 0.144 0.146 0.148 0.15 0.152 0.154 0.156 0.158 0.16 0.162 0.164 0.166 0.168 0.17 0.172 0.174 0.176 0.178 0.18 0.182 0.184 0.186 0.188 0.19 0.192 0.194 0.196 0.198 0.2 0.202 0.204 0.206 0.208 0.21 0.212 0.214 0.216 0.218 0.22 0.222 0.224 0.226 0.228 0.23 0.232 0.234 0.236 0.238 0.24 0.242 0.244 0.246 0.248 0.25]
      | sbobj.Groups(6).Signals(3).YData = [-1 1 -1 1 -1 1 -1 0 0 0 1 -1 1 0 -1 1 -1 1 0 0 1 -1 1 -1 1 -1 1 -1 0 0 0 1 -1 1 0 -1 1 -1 1 0 0 1 -1 1 -1 1 -1 1 -1 0 0 0 1 -1 1 0 -1 1 -1 1 0 0 1 -1 1 -1 1 -1 1 -1 0 0 0 1 -1 1 0 -1 1 -1 1 0 0 1 -1 1 -1 1 -1 1 -1 0 0 0 1 -1 1 0 -1 1 -1 1 0 0 1 -1 1 -1 1 -1 1 -1 0 0 0 1 -1 1 0 -1 1 -1 1 0 0 1]
      | sbobj.Groups(6).TimeRange = [0 0.25]
      | sbobj.Groups(7).Name = 'RollCntr>255'
      | sbobj.Groups(7).Signals(1).Name = 'MotAg2Sin'
      | sbobj.Groups(7).Signals(1).XData = [0 0.002 0.004 0.006 0.008 0.01 0.012 0.014 0.016 0.018 0.02 0.022 ... (501 elements, 1x501)]
      | sbobj.Groups(7).Signals(1).YData = [0 2.5 4.5 5 4.5 2.5 0 2.5 4.5 5 4.5 2.5 0 2.5 4.5 5 4.5 2.5 0 2.5 4.5 5 4.5 2.5 0 2.5 4.5 5 4.5 2.5 0 2.5 4.5 5 4.5 2.5 0 2.5 4.5 5 4.5 2.5 0 2.5 4.5 5 4.5 2.5 0 2.5 4.5 5 4.5 2.5 0 2.5 4.5 5 4.5 2.5 0 2.5 4.5 5 4.5 2.5 0 2.5 4.5 5 4.5 2.5 0 2.5 4.5 5 4.5 2.5 0 2.5 4.5 5 4.5 2.5 0 2.5 4.5 5 4.5 2.5 0 2.5 4.5 5 4.5 2.5 0 2.5 4.5 5 4.5 2.5 0 2.5 4.5 5 4.5 2.5 0 2.5 4.5 5 4.5 2.5 0 2.5 4.5 5 4.5 2.5 0 2.5 4.5 5 4.5 2.5 0 2.5 4.5 5 4.5 2.5 0 2.5 4.5 5 4.5 2.5 0 2.5 4.5 5 4.5 2.5 0 2.5 4.5 5 4.5 2.5 0 2.5 4.5 5 4.5 2.5 0 2.5 4.5 5 4.5 2.5 0 2.5 4.5 5 4.5 2.5 0 2.5 4.5 5 4.5 2.5 0 2.5 4.5 5 4.5 2.5 0 2.5 4.5 5 4.5 2.5 0 2.5 4.5 5 4.5 2.5 0 2.5 4.5 5 4.5 2.5 0 2.5 4.5 5 4.5 2.5 0 2.5 4.5 5 4.5 2.5 0 2.5 4.5 5 4.5 2.5 0 2.5 4.5 5 4.5 2.5 0 2.5 4.5 5 4.5 2.5 0 2.5 4.5 5 4.5 2.5 0 2.5 4.5 5 4.5 2.5 0 2.5 4.5 5 4.5 2.5 0 2.5 4.5 5 4.5 2.5 0 2.5 4.5 5 4.5 2.5 0 2.5 4.5 5 4.5 2.5 0 2.5 4.5 5 4.5 2.5 0 2.5 4.5 5 4.5 2.5 0 2.5 4.5 5 4.5 2.5 0 2.5 4.5 5 4.5 2.5 0 2.5 4.5 5 4.5 2.5 0 2.5 4.5 5 4.5 2.5 0 2.5 4.5 5 4.5 2.5 0 2.5 4.5 5 4.5 2.5 0 2.5 4.5 5 4.5 2.5 0 2.5 4.5 5 4.5 2.5 0 2.5 4.5 5 4.5 2.5 0 2.5 4.5 5 4.5 2.5 0 2.5 4.5 5 4.5 2.5 0 2.5 4.5 5 4.5 2.5 0 2.5 4.5 5 4.5 2.5 0 2.5 4.5 5 4.5 2.5 0 2.5 4.5 5 4.5 2.5 0 2.5 4.5 5 4.5 2.5 0 2.5 4.5 5 0 2.5 4.5 5 4.5 2.5 0 2.5 4.5 5 4.5 2.5 0 2.5 4.5 5 4.5 2.5 0 2.5 4.5 5 4.5 2.5 0 2.5 4.5 5 4.5 2.5 0 2.5 4.5 5 4.5 2.5 0 2.5 4.5 5 4.5 2.5 0 2.5 4.5 5 4.5 2.5 0 2.5 4.5 5 4.5 2.5 0 2.5 4.5 5 4.5 2.5 0 2.5 4.5 5 4.5 2.5 0 2.5 4.5 5 4.5 2.5 0 2.5 4.5 5 4.5 2.5 0 2.5 4.5 5 4.5 2.5 0 2.5 4.5 5 4.5 2.5 0 2.5 4.5 5 4.5 2.5 0 2.5 4.5 5 4.5 2.5 0 2.5 4.5 5 4.5 2.5 0 2.5 4.5 5 4.5 2.5 0 2.5 4.5 5 4.5 2.5 0 2.5 4.5 5 4.5]
      | sbobj.Groups(7).Signals(2).Name = 'MotAg2Cos'
      | sbobj.Groups(7).Signals(2).XData = [0 0.002 0.004 0.006 0.008 0.01 0.012 0.014 0.016 0.018 0.02 0.022 ... (501 elements, 1x501)]
      | sbobj.Groups(7).Signals(2).YData = [5 4.5 2.5 0 2.5 4.5 5 4.5 2.5 0 2.5 4.5 5 4.5 2.5 0 2.5 4.5 5 4.5 2.5 0 2.5 4.5 5 4.5 2.5 0 2.5 4.5 5 4.5 2.5 0 2.5 4.5 5 4.5 2.5 0 2.5 4.5 5 4.5 2.5 0 2.5 4.5 5 4.5 2.5 0 2.5 4.5 5 4.5 2.5 0 2.5 4.5 5 4.5 2.5 0 2.5 4.5 5 4.5 2.5 0 2.5 4.5 5 4.5 2.5 0 2.5 4.5 5 4.5 2.5 0 2.5 4.5 5 4.5 2.5 0 2.5 4.5 5 4.5 2.5 0 2.5 4.5 5 4.5 2.5 0 2.5 4.5 5 4.5 2.5 0 2.5 4.5 5 4.5 2.5 0 2.5 4.5 5 4.5 2.5 0 2.5 4.5 5 4.5 2.5 0 2.5 4.5 5 4.5 2.5 0 2.5 4.5 5 4.5 2.5 0 2.5 4.5 5 4.5 2.5 0 2.5 4.5 5 4.5 2.5 0 2.5 4.5 5 4.5 2.5 0 2.5 4.5 5 4.5 2.5 0 2.5 4.5 5 4.5 2.5 0 2.5 4.5 5 4.5 2.5 0 2.5 4.5 5 4.5 2.5 0 2.5 4.5 5 4.5 2.5 0 2.5 4.5 5 4.5 2.5 0 2.5 4.5 5 4.5 2.5 0 2.5 4.5 5 4.5 2.5 0 2.5 4.5 5 4.5 2.5 0 2.5 4.5 5 4.5 2.5 0 2.5 4.5 5 4.5 2.5 0 2.5 4.5 5 4.5 2.5 0 2.5 4.5 5 4.5 2.5 0 2.5 4.5 5 4.5 2.5 0 2.5 4.5 5 4.5 2.5 0 2.5 4.5 5 4.5 2.5 0 2.5 4.5 5 4.5 2.5 0 2.5 4.5 5 4.5 2.5 0 2.5 4.5 5 4.5 2.5 0 2.5 4.5 5 4.5 2.5 0 2.5 4.5 5 4.5 2.5 0 2.5 4.5 5 4.5 2.5 0 2.5 4.5 5 4.5 2.5 0 2.5 4.5 5 4.5 2.5 0 2.5 4.5 5 4.5 2.5 0 2.5 4.5 5 4.5 2.5 0 2.5 4.5 5 4.5 2.5 0 2.5 4.5 5 4.5 2.5 0 2.5 4.5 5 4.5 2.5 0 2.5 4.5 5 4.5 2.5 0 2.5 4.5 5 4.5 2.5 0 2.5 4.5 5 4.5 2.5 0 2.5 4.5 5 4.5 2.5 0 2.5 4.5 5 4.5 2.5 0 2.5 4.5 5 4.5 2.5 0 2.5 4.5 5 4.5 2.5 0 2.5 4.5 5 4.5 2.5 0 5 4.5 2.5 0 2.5 4.5 5 4.5 2.5 0 2.5 4.5 5 4.5 2.5 0 2.5 4.5 5 4.5 2.5 0 2.5 4.5 5 4.5 2.5 0 2.5 4.5 5 4.5 2.5 0 2.5 4.5 5 4.5 2.5 0 2.5 4.5 5 4.5 2.5 0 2.5 4.5 5 4.5 2.5 0 2.5 4.5 5 4.5 2.5 0 2.5 4.5 5 4.5 2.5 0 2.5 4.5 5 4.5 2.5 0 2.5 4.5 5 4.5 2.5 0 2.5 4.5 5 4.5 2.5 0 2.5 4.5 5 4.5 2.5 0 2.5 4.5 5 4.5 2.5 0 2.5 4.5 5 4.5 2.5 0 2.5 4.5 5 4.5 2.5 0 2.5 4.5 5 4.5 2.5 0 2.5 4.5 5 4.5 2.5 0 2.5 4.5 5 4.5 2.5 0 2.5]
      | sbobj.Groups(7).Signals(3).Name = 'MotAgMecl2Polarity'
      | sbobj.Groups(7).Signals(3).XData = [0 0.002 0.004 0.006 0.008 0.01 0.012 0.014 0.016 0.018 0.02 0.022 ... (501 elements, 1x501)]
      | sbobj.Groups(7).Signals(3).YData = [-1 1 -1 1 -1 1 -1 0 0 0 1 -1 1 0 -1 1 -1 1 0 0 1 -1 1 -1 1 -1 1 -1 0 0 0 1 -1 1 0 -1 1 -1 1 0 0 1 -1 1 -1 1 -1 1 -1 0 0 0 1 -1 1 0 -1 1 -1 1 0 0 1 -1 1 -1 1 -1 1 -1 0 0 0 1 -1 1 0 -1 1 -1 1 0 0 1 -1 1 -1 1 -1 1 -1 0 0 0 1 -1 1 0 -1 1 -1 1 0 0 1 -1 1 -1 1 -1 1 -1 0 0 0 1 -1 1 0 -1 1 -1 1 0 0 1 -1 1 -1 1 -1 1 -1 0 0 0 1 -1 1 0 -1 1 -1 1 0 0 1 -1 1 -1 1 -1 1 -1 0 0 0 1 -1 1 0 -1 1 -1 1 0 0 1 -1 1 -1 1 -1 1 -1 0 0 0 1 -1 1 0 -1 1 -1 1 0 0 1 -1 1 -1 1 -1 1 -1 0 0 0 1 -1 1 0 -1 1 -1 1 0 0 1 -1 1 -1 1 -1 1 -1 0 0 0 1 -1 1 0 -1 1 -1 1 0 0 1 -1 1 -1 1 -1 1 -1 0 0 0 1 -1 1 0 -1 1 -1 1 0 0 1 -1 1 -1 1 -1 1 -1 0 0 0 1 -1 1 0 -1 1 -1 1 0 0 1 -1 1 -1 1 -1 1 -1 0 0 0 1 -1 1 0 -1 1 -1 1 0 0 1 -1 1 -1 1 -1 1 -1 0 0 0 1 -1 1 0 -1 1 -1 1 0 0 1 -1 1 -1 1 -1 1 -1 0 0 0 1 -1 1 0 -1 1 -1 1 0 0 1 -1 1 -1 1 -1 1 -1 0 0 0 1 -1 1 0 -1 1 -1 1 0 0 1 -1 1 -1 1 -1 1 -1 0 0 0 1 -1 1 0 -1 1 -1 1 0 -1 1 -1 1 -1 1 -1 0 0 0 1 -1 1 0 -1 1 -1 1 0 0 1 -1 1 -1 1 -1 1 -1 0 0 0 1 -1 1 0 -1 1 -1 1 0 0 1 -1 1 -1 1 -1 1 -1 0 0 0 1 -1 1 0 -1 1 -1 1 0 0 1 -1 1 -1 1 -1 1 -1 0 0 0 1 -1 1 0 -1 1 -1 1 0 0 1 -1 1 -1 1 -1 1 -1 0 0 0 1 -1 1 0 -1 1 -1 1 0 0 1 -1 1 -1 1 -1 1 -1 0 0 0 1 -1 1 0 -1 1 -1 1 0 0]
      | sbobj.Groups(7).TimeRange = [0 1]
      | sbobj.Groups(8).Name = 'NoFault'
      | sbobj.Groups(8).Signals(1).Name = 'MotAg2Sin'
      | sbobj.Groups(8).Signals(1).XData = [0 1]
      | sbobj.Groups(8).Signals(1).YData = [2.5 2.5]
      | sbobj.Groups(8).Signals(2).Name = 'MotAg2Cos'
      | sbobj.Groups(8).Signals(2).XData = [0 1]
      | sbobj.Groups(8).Signals(2).YData = [2 2]
      | sbobj.Groups(8).Signals(3).Name = 'MotAgMecl2Polarity'
      | sbobj.Groups(8).Signals(3).XData = [0 0.002 0.004 0.006 0.008 0.01 0.012 0.014 0.016 0.018 0.02 0.022 0.024 0.026 0.028 0.03 0.032 0.034 0.036 0.038 0.04 1]
      | sbobj.Groups(8).Signals(3).YData = [-1 1 -1 1 -1 1 -1 0 0 0 1 -1 1 0 -1 1 -1 1 0 0 1 1]
      | sbobj.Groups(8).TimeRange = [0 1]
  MotAg2Sin : Outport
  MotAg2Cos : Outport  Tag=STV Outport  Port=2
  MotAgMecl2Polarity : Outport  Tag=STV Outport  Port=3
  wires:
  Demux/1 -> MotAg2Sin/1
  FromWs/1 -> Demux/1
  Demux/2 -> MotAg2Cos/1
  Demux/3 -> MotAgMecl2Polarity/1

== system ES241A_MotAg2Meas/Write_Trigger ==
  Enable : EnablePort
  Function-Call Generator1 : simulink/Ports & Subsystems/Function-Call Generator  sample_time=0.002  numberOfIterations=1
  Out1 : Outport
  wires:
  Function-Call Generator1/1 -> Out1/1

== system ES241A_MotAg2Meas/MotAg2Meas/CopyRight2 ==

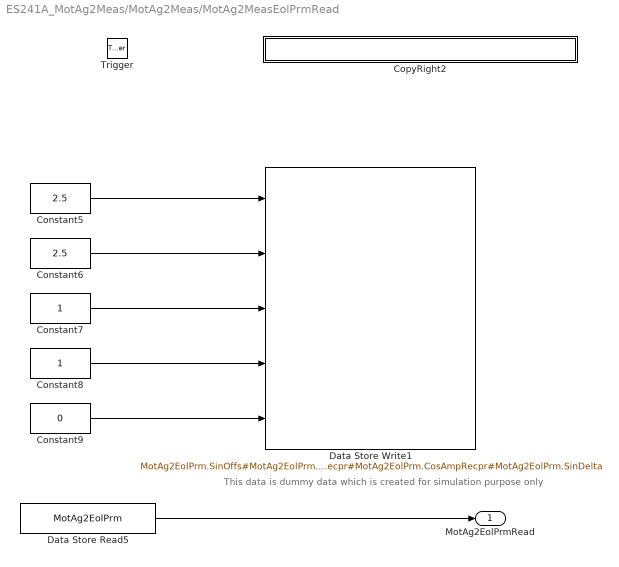
== system ES241A_MotAg2Meas/MotAg2Meas/MotAg2MeasEolPrmRead ==
  note: This data is dummy data which is created for simulation purpose only
  Trigger : TriggerPort  TriggerType=function-call  PortDimensions=1
  Constant5 : Constant  Value=2.5  OutDataTypeStr=single
  Constant6 : Constant  Value=2.5  OutDataTypeStr=single
  Constant7 : Constant  OutDataTypeStr=single
  Constant8 : Constant  OutDataTypeStr=single
  Constant9 : Constant  Value=0  OutDataTypeStr=single
  CopyRight2 : Subsystem  Description=|  mask(Copyright Information){none=on}
      | Copyright info block.                                               
      |                                                                     
      | Place copyright information at the top of every subsystem in design.
      mask prompts: none "No parameters"
      mask help: Place copyright information at the top of every subsystem in design.
      mask Display:
      | NxtrConf = 'Nexteer Confidential';
      | 
      | sys = bdroot; %handle for the current model ("system")
      | first = get_param(sys,'Created');
      | first = first(end-3:end);  %year is last four digits
      | 
      | last = get_param(sys,'LastModifiedDate');
      | if isempty(last)
      |     last = datestr(now,'yyyy');
      | else
      |     last = last(end-3:end);
      | end
      | 
      | if strcmp(first,last)
      |     fprintf('%s -- Copyright %s Nexteer',NxtrConf,first)
      | else
      |     fprintf('%s -- %s%s- %s Nexteer',NxtrConf,char(169),first,last)
      | end
  Data Store Read5 : DataStoreRead  DataStoreName=MotAg2EolPrm
  Data Store Write1 : DataStoreWrite  DataStoreName=MotAg2EolPrm  DataStoreElements=MotAg2EolPrm.SinOffs#MotAg2EolPrm.CosOffs#MotAg2EolPrm.SinAmpRecpr#MotAg2EolPrm.CosAmpRecpr#MotAg2EolPrm.SinDelta
  MotAg2EolPrmRead : Outport  OutDataTypeStr=Bus: MotAgMeasEolPrmRec1
  wires:
  Constant5/1 -> Data Store Write1/1
  Constant6/1 -> Data Store Write1/2
  Constant9/1 -> Data Store Write1/5
  Constant8/1 -> Data Store Write1/4
  Constant7/1 -> Data Store Write1/3
  Data Store Read5/1 -> MotAg2EolPrmRead/1

== system ES241A_MotAg2Meas/MotAg2Meas/MotAg2MeasEolPrmWr ==
  MotAg2SinCosData : Inport
  Trigger : TriggerPort  TriggerType=function-call  PortDimensions=1
  Constant1 : Constant  Value=true  OutDataTypeStr=boolean
      settings: AttributesFormatString=%<OutDataTypeStr>
  Copyright2 : Subsystem  Description=|  mask(Copyright Information){none=on}
      | Copyright info block.                                               
      |                                                                     
      | Place copyright information at the top of every subsystem in design.
      mask prompts: none "No parameters"
      mask help: Place copyright information at the top of every subsystem in design.
      mask Display:
      | NxtrConf = 'Nexteer Confidential';
      | 
      | sys = bdroot; %handle for the current model ("system")
      | first = get_param(sys,'Created');
      | if(isempty(first))
      |     first = datestr(now,'yyyy');
      | else
      |     first = first(end-3:end);  %year is last four digits
      | end
      | 
      | last = get_param(sys,'LastModifiedDate');
      | if isempty(last)
      |     last = datestr(now,'yyyy');
      | else
      |     last = last(end-3:end);
      | end
      | 
      | if strcmp(first,last)
      |     fprintf('%s\nCopyright  %s Nexteer',NxtrConf,first);
      | else
      |     fprintf('%s\n%s%s-%s Nexteer',NxtrConf,char(169),first,last);
      | end
  Data Store Write : DataStoreWrite  DataStoreName=MotAg2EolPrm
  MotAg2EolPrm_SetRamBlockStatus : Subsystem
  wires:
  MotAg2SinCosData/1 -> Data Store Write/1
  Constant1/1 -> MotAg2EolPrm_SetRamBlockStatus/1(BlockChanged)

== system ES241A_MotAg2Meas/MotAg2Meas/MotAg2MeasInit1 ==
  function : TriggerPort  TriggerType=function-call
  CopyRight2 : Subsystem  Description=|  mask(Copyright Information){none=on}
      | Copyright info block.                                               
      |                                                                     
      | Place copyright information at the top of every subsystem in design.
      mask prompts: none "No parameters"
      mask help: Place copyright information at the top of every subsystem in design.
      mask Display:
      | NxtrConf = 'Nexteer Confidential';
      | 
      | sys = bdroot; %handle for the current model ("system")
      | first = get_param(sys,'Created');
      | first = first(end-3:end);  %year is last four digits
      | 
      | last = get_param(sys,'LastModifiedDate');
      | if isempty(last)
      |     last = datestr(now,'yyyy');
      | else
      |     last = last(end-3:end);
      | end
      | 
      | if strcmp(first,last)
      |     fprintf('%s -- Copyright %s Nexteer',NxtrConf,first)
      | else
      |     fprintf('%s -- %s%s- %s Nexteer',NxtrConf,char(169),first,last)
      | end
  If : If  IfExpression=u1 == 0
  MotAg2EolPrm_GetErrorStatus : Subsystem  RequirementInfo={'linktype_rmi_doors' '0000cf65 (/E-STEER Core/SubSystem Specifications/Electrical Actuator/Control Module/FDD Module Requirements/EA4/ES241A_MotAg2Meas)' '#ES241A_140' 'true' 'REQ: ES241A_140' '' } %GIDa_4f88992a_8b37_4448_b960_f80c6530b4b6  TreatAsAtomicUnit=on
  NVM_NOK : Subsystem  RequirementInfo={'linktype_rmi_doors' '0000cf65 (/E-STEER Core/SubSystem Specifications/Electrical Actuator/Control Module/FDD Module Requirements/EA4/ES241A_MotAg2Meas)' '#ES241A_141' 'true' 'REQ: ES241A_141' '' } %GIDa_30aca007_0271_4e5d_a94c_7338dfdad936  TreatAsAtomicUnit=on
  NVM_Ok : Subsystem  TreatAsAtomicUnit=on
  wires:
  MotAg2EolPrm_GetErrorStatus/1(RequestResultPtr) -> If/1
  If/1 -> NVM_Ok/Action
  If/2 -> NVM_NOK/Action

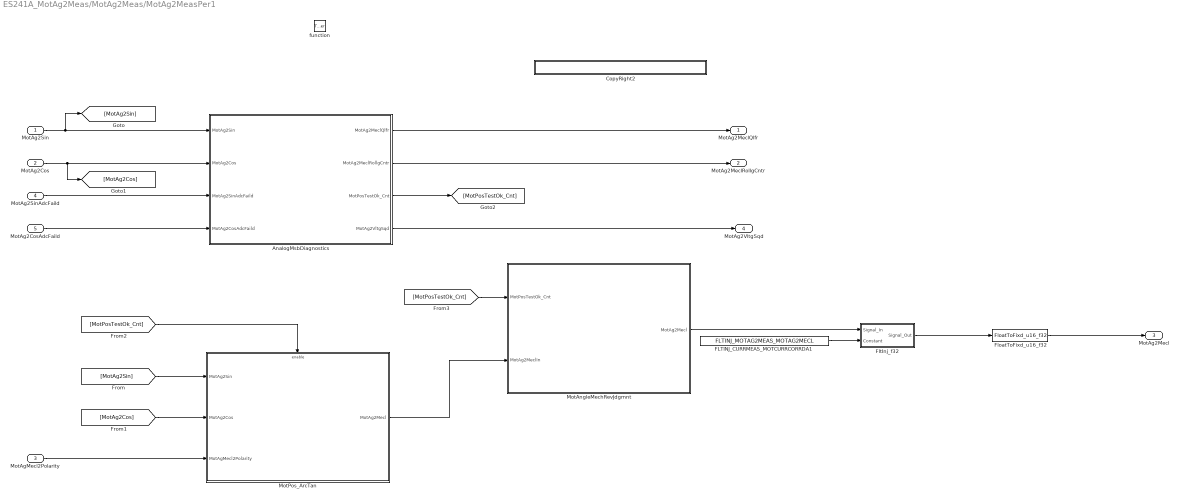
== system ES241A_MotAg2Meas/MotAg2Meas/MotAg2MeasPer1 ==
  MotAg2Sin : Inport
  MotAg2Cos : Inport  Port=2
  MotAgMecl2Polarity : Inport  Port=3
  MotAg2SinAdcFaild : Inport  RequirementInfo={} %GIDa_58f11d78_1898_4a56_85a8_3c263e97ba5e  Port=4
  MotAg2CosAdcFaild : Inport  RequirementInfo={} %GIDa_6239d747_cd2d_45c0_94f0_fc30ee06b788  Port=5
  function : TriggerPort  TriggerType=function-call
  AnalogMsbDiagnostics : Subsystem  RequirementInfo={'linktype_rmi_doors' '0000cf65 (/E-STEER Core/SubSystem Specifications/Electrical Actuator/Control Module/FDD Module Requirements/EA4/ES241A_MotAg2Meas)' '#ES241A_139' 'true' 'REQ: ES241A_139' '' ; 'linktype_rmi_doors' '0000cf65 (/E-STEER Core/SubSystem Specifications/Electrical Actuator/Control Module/FDD Module Requirements/EA4/ES241A_MotAg2Meas)' '#ES241A_131' 'true' 'REQ: ES241A_131' '' } %GIDa_f21488b9_17b1_4c0d_818a_1298dc68aed3
  CopyRight2 : Subsystem  Description=|  mask(Copyright Information){none=on}
      | Copyright info block.                                               
      |                                                                     
      | Place copyright information at the top of every subsystem in design.
      mask prompts: none "No parameters"
      mask help: Place copyright information at the top of every subsystem in design.
      mask Display:
      | NxtrConf = 'Nexteer Confidential';
      | 
      | sys = bdroot; %handle for the current model ("system")
      | first = get_param(sys,'Created');
      | if(isempty(first))
      |     first = datestr(now,'yyyy');
      | else
      |     first = first(end-3:end);  %year is last four digits
      | end
      | 
      | last = get_param(sys,'LastModifiedDate');
      | if isempty(last)
      |     last = datestr(now,'yyyy');
      | else
      |     last = last(end-3:end);
      | end
      | 
      | if strcmp(first,last)
      |     fprintf('%s -- Copyright %s Nexteer',NxtrConf,first)
      | else
      |     fprintf('%s -- %s%s- %s Nexteer',NxtrConf,char(169),first,last)
      | end
  FLTINJ_CURRMEAS_MOTCURRCORRDA1 : Constant  Value=FLTINJ_MOTAG2MEAS_MOTAG2MECL
  FloatToFixd_u16_f32 : FloatToFixd/FloatToFixd_u16_f32  Param1=16
  FltInj_f32 : Subsystem  RequirementInfo={'linktype_rmi_doors' '0000cf65 (/E-STEER Core/SubSystem Specifications/Electrical Actuator/Control Module/FDD Module Requirements/EA4/ES241A_MotAg2Meas)' '#ES241A_143' 'true' 'REQ: ES241A_143' '' } %GIDa_cb902eb8_44d0_4b6b_8c02_d7b413fb0ac3  TreatAsAtomicUnit=on  VariantControl=FltInj_sim  mask(Fault_Injection){}
      mask help: Fault Injection is a simulation only block for EA3 programs.
  MotAngleMechRevJdgmnt : Subsystem  RequirementInfo={'linktype_rmi_doors' '0000cf65 (/E-STEER Core/SubSystem Specifications/Electrical Actuator/Control Module/FDD Module Requirements/EA4/ES241A_MotAg2Meas)' '#ES241A_139' 'true' 'REQ: ES241A_139' '' } %GIDa_5d8fadd9_6f5e_4fdb_aed8_790cd455caed
  MotPos_ArcTan : Subsystem  RequirementInfo={} %GIDa_e2481928_7d11_4a85_9792_bf58e36239d5  TreatAsAtomicUnit=on
  MotAg2MeclQlfr : Outport
  MotAg2MeclRollgCntr : Outport  Port=2
  MotAg2Mecl : Outport  Port=3
  MotAg2VltgSqd : Outport  Port=4
  wires:
  MotAg2Sin/1 -> [MotAg2Sin], AnalogMsbDiagnostics/1(MotAg2Sin)
  MotAg2Cos/1 -> [MotAg2Cos], AnalogMsbDiagnostics/2(MotAg2Cos)
  MotAgMecl2Polarity/1 -> MotPos_ArcTan/3(MotAgMecl2Polarity)
  [MotAg2Cos] -> MotPos_ArcTan/2(MotAg2Cos)
  AnalogMsbDiagnostics/1(MotAg2MeclQlfr) -> MotAg2MeclQlfr/1
  AnalogMsbDiagnostics/2(MotAg2MeclRollgCntr) -> MotAg2MeclRollgCntr/1
  MotPos_ArcTan/1(MotAg2Mecl) -> MotAngleMechRevJdgmnt/2(MotAg2MeclIn)
  MotAngleMechRevJdgmnt/1(MotAg2Mecl) -> FltInj_f32/1(Signal_In)
  AnalogMsbDiagnostics/3(MotPosTestOk_Cnt) -> [MotPosTestOk_Cnt]
  [MotPosTestOk_Cnt] -> MotPos_ArcTan/Enable
  [MotPosTestOk_Cnt] -> MotAngleMechRevJdgmnt/1(MotPosTestOk_Cnt)
  [MotAg2Sin] -> MotPos_ArcTan/1(MotAg2Sin)
  FLTINJ_CURRMEAS_MOTCURRCORRDA1/1 -> FltInj_f32/2(Constant)
  FltInj_f32/1(Signal_Out) -> FloatToFixd_u16_f32/1
  FloatToFixd_u16_f32/1 -> MotAg2Mecl/1
  MotAg2SinAdcFaild/1 -> AnalogMsbDiagnostics/3(MotAg2SinAdcFaild)
  MotAg2CosAdcFaild/1 -> AnalogMsbDiagnostics/4(MotAg2CosAdcFaild)
  AnalogMsbDiagnostics/4(MotAg2VltgSqd) -> MotAg2VltgSqd/1

== system ES241A_MotAg2Meas/MotAg2Meas/MotAg2MeasEolPrmRead/CopyRight2 ==

== system ES241A_MotAg2Meas/MotAg2Meas/MotAg2MeasEolPrmWr/Copyright2 ==

== system ES241A_MotAg2Meas/MotAg2Meas/MotAg2MeasEolPrmWr/MotAg2EolPrm_SetRamBlockStatus ==
  note: This is the block representing the client call
  BlockChanged : Inport
  Terminator : Terminator
  wires:
  BlockChanged/1 -> Terminator/1

== system ES241A_MotAg2Meas/MotAg2Meas/MotAg2MeasInit1/CopyRight2 ==

== system ES241A_MotAg2Meas/MotAg2Meas/MotAg2MeasInit1/MotAg2EolPrm_GetErrorStatus ==
  note: 0 simulated for modeling purposes,
      | actual value returned by NVM.  Non-zero return indicates
      | failure in storage/retrievial of NVM.
  Constant : Constant  Value=0
  CopyRight2 : Subsystem  Description=|  mask(Copyright Information){none=on}
      | Copyright info block.                                               
      |                                                                     
      | Place copyright information at the top of every subsystem in design.
      mask prompts: none "No parameters"
      mask help: Place copyright information at the top of every subsystem in design.
      mask Display:
      | NxtrConf = 'Nexteer Confidential';
      | 
      | sys = bdroot; %handle for the current model ("system")
      | first = get_param(sys,'Created');
      | first = first(end-3:end);  %year is last four digits
      | 
      | last = get_param(sys,'LastModifiedDate');
      | if isempty(last)
      |     last = datestr(now,'yyyy');
      | else
      |     last = last(end-3:end);
      | end
      | 
      | if strcmp(first,last)
      |     fprintf('%s -- Copyright %s Nexteer',NxtrConf,first)
      | else
      |     fprintf('%s -- %s%s- %s Nexteer',NxtrConf,char(169),first,last)
      | end
  RequestResultPtr : Outport
  wires:
  Constant/1 -> RequestResultPtr/1

== system ES241A_MotAg2Meas/MotAg2Meas/MotAg2MeasInit1/NVM_NOK ==
  note: In the event of a NVM failure
      | zero out the whole shadow ram image
  Action Port : ActionPort  ActionType=else
  Constant{1..5} (5 alike) : Constant  Value=0  OutDataTypeStr=Inherit: Inherit via back propagation
  CopyRight2 : Subsystem  Description=|  mask(Copyright Information){none=on}
      | Copyright info block.                                               
      |                                                                     
      | Place copyright information at the top of every subsystem in design.
      mask prompts: none "No parameters"
      mask help: Place copyright information at the top of every subsystem in design.
      mask Display:
      | NxtrConf = 'Nexteer Confidential';
      | 
      | sys = bdroot; %handle for the current model ("system")
      | first = get_param(sys,'Created');
      | first = first(end-3:end);  %year is last four digits
      | 
      | last = get_param(sys,'LastModifiedDate');
      | if isempty(last)
      |     last = datestr(now,'yyyy');
      | else
      |     last = last(end-3:end);
      | end
      | 
      | if strcmp(first,last)
      |     fprintf('%s -- Copyright %s Nexteer',NxtrConf,first)
      | else
      |     fprintf('%s -- %s%s- %s Nexteer',NxtrConf,char(169),first,last)
      | end
  Data Store Write2 : DataStoreWrite  DataStoreName=MotAg2EolPrm  DataStoreElements=MotAg2EolPrm.SinOffs#MotAg2EolPrm.CosOffs#MotAg2EolPrm.SinAmpRecpr#MotAg2EolPrm.CosAmpRecpr#MotAg2EolPrm.SinDelta
  wires:
  Constant1/1 -> Data Store Write2/1
  Constant2/1 -> Data Store Write2/2
  Constant4/1 -> Data Store Write2/4
  Constant3/1 -> Data Store Write2/3
  Constant5/1 -> Data Store Write2/5

== system ES241A_MotAg2Meas/MotAg2Meas/MotAg2MeasInit1/NVM_Ok ==
  note: ***********  This block is for simulation purposes only *******************8
      |
      | The module should use the shadow RAM image
  Action Port : ActionPort  ActionType=then
  Constant : Constant  Value=2.5  OutDataTypeStr=single
  Constant1 : Constant  Value=2.5  OutDataTypeStr=single
  Constant2 : Constant  OutDataTypeStr=single
  Constant3 : Constant  OutDataTypeStr=single
  Constant4 : Constant  Value=0  OutDataTypeStr=single
  CopyRight2 : Subsystem  Description=|  mask(Copyright Information){none=on}
      | Copyright info block.                                               
      |                                                                     
      | Place copyright information at the top of every subsystem in design.
      mask prompts: none "No parameters"
      mask help: Place copyright information at the top of every subsystem in design.
      mask Display:
      | NxtrConf = 'Nexteer Confidential';
      | 
      | sys = bdroot; %handle for the current model ("system")
      | first = get_param(sys,'Created');
      | first = first(end-3:end);  %year is last four digits
      | 
      | last = get_param(sys,'LastModifiedDate');
      | if isempty(last)
      |     last = datestr(now,'yyyy');
      | else
      |     last = last(end-3:end);
      | end
      | 
      | if strcmp(first,last)
      |     fprintf('%s -- Copyright %s Nexteer',NxtrConf,first)
      | else
      |     fprintf('%s -- %s%s- %s Nexteer',NxtrConf,char(169),first,last)
      | end
  Data Store Write1 : DataStoreWrite  DataStoreName=MotAg2EolPrm  DataStoreElements=MotAg2EolPrm.SinOffs#MotAg2EolPrm.CosOffs#MotAg2EolPrm.SinAmpRecpr#MotAg2EolPrm.CosAmpRecpr#MotAg2EolPrm.SinDelta
  wires:
  Constant/1 -> Data Store Write1/1
  Constant1/1 -> Data Store Write1/2
  Constant4/1 -> Data Store Write1/5
  Constant3/1 -> Data Store Write1/4
  Constant2/1 -> Data Store Write1/3

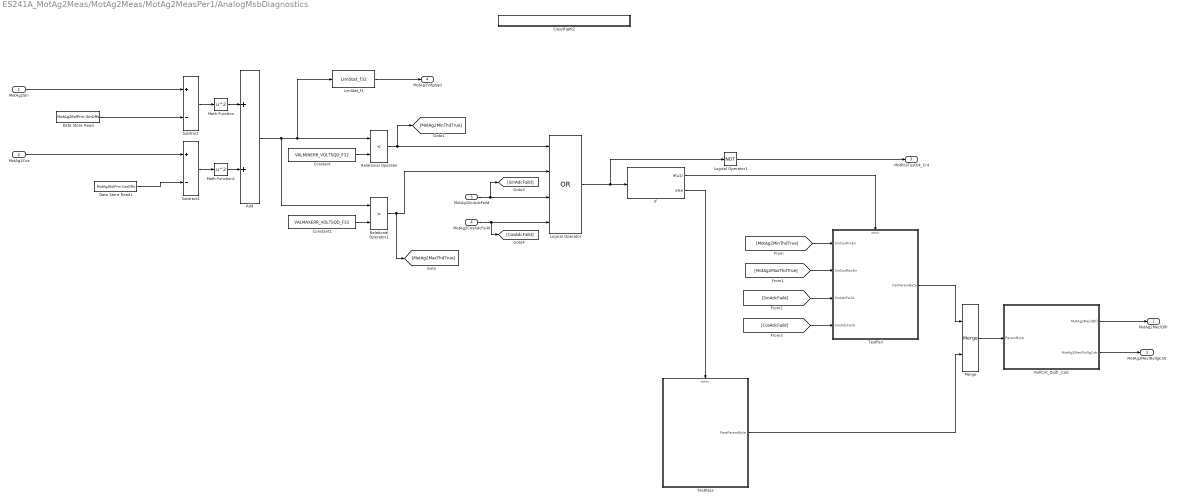
== system ES241A_MotAg2Meas/MotAg2Meas/MotAg2MeasPer1/AnalogMsbDiagnostics ==
  MotAg2Sin : Inport  RequirementInfo={} %GIDa_c492a74e_e9d8_4350_a9f2_7aaf25ec4f85
  MotAg2Cos : Inport  RequirementInfo={} %GIDa_f563396c_c31e_448d_9334_0b07e8708bb7  Port=2
  MotAg2SinAdcFaild : Inport  RequirementInfo={} %GIDa_12d9194d_b121_452c_a63d_2c04aa0c4a74  Port=3
  MotAg2CosAdcFaild : Inport  RequirementInfo={} %GIDa_4f2bf034_ef8a_4b03_9482_45ff9ee3c56d  Port=4
  Add : Sum  RequirementInfo={} %GIDa_42d846aa_1305_433b_abbb_13ea02e99d63
  Constant : Constant  RequirementInfo={} %GIDa_475dfb7c_498a_4985_b491_c529d057db80  Value=VALMINERR_VOLTSQD_F32
  Constant1 : Constant  RequirementInfo={} %GIDa_8b43fc00_2e57_4672_a45d_13f5fb16af82  Value=VALMAXERR_VOLTSQD_F32
  CopyRight2 : Subsystem  Description=|  mask(Copyright Information){none=on}
      | Copyright info block.                                               
      |                                                                     
      | Place copyright information at the top of every subsystem in design.
      mask prompts: none "No parameters"
      mask help: Place copyright information at the top of every subsystem in design.
      mask Display:
      | NxtrConf = 'Nexteer Confidential';
      | 
      | sys = bdroot; %handle for the current model ("system")
      | first = get_param(sys,'Created');
      | if(isempty(first))
      |     first = datestr(now,'yyyy');
      | else
      |     first = first(end-3:end);  %year is last four digits
      | end
      | 
      | last = get_param(sys,'LastModifiedDate');
      | if isempty(last)
      |     last = datestr(now,'yyyy');
      | else
      |     last = last(end-3:end);
      | end
      | 
      | if strcmp(first,last)
      |     fprintf('%s -- Copyright %s Nexteer',NxtrConf,first)
      | else
      |     fprintf('%s -- %s%s- %s Nexteer',NxtrConf,char(169),first,last)
      | end
  Data Store Read : DataStoreRead  DataStoreName=MotAg2EolPrm  DataStoreElements=MotAg2EolPrm.SinOffs
  Data Store Read1 : DataStoreRead  DataStoreName=MotAg2EolPrm  DataStoreElements=MotAg2EolPrm.CosOffs
  If : If  IfExpression=u1
  LimStat_f1 : NxtrLim/LimStat_f32  RequirementInfo={'linktype_rmi_doors' '0000cf65 (/E-STEER Core/SubSystem Specifications/Electrical Actuator/Control Module/FDD Module Requirements/EA4/ES241A_MotAg2Meas)' '#ES241A_16' 'true' 'REQ: ES241A_16' '' } %GIDa_141367ea_ace8_40b3_a4b6_af866b452f13  LoLim=MotAg2VltgSqd.EngMin  HiLim=MotAg2VltgSqd.EngMax
      settings: AttributesFormatString=|
      | Low Limit: %<LoLim>
      | High Limit:%<HiLim>
  Logical Operator : Logic  RequirementInfo={} %GIDa_291c91d4_1ffd_47bd_894d_802f0d1c9a8c  Operator=OR  Inputs=4  AllPortsSameDT=off  OutDataTypeStr=boolean
  Logical Operator1 : Logic  Operator=NOT  AllPortsSameDT=off  OutDataTypeStr=boolean
  Math Function : Math  RequirementInfo={} %GIDa_1e42a42a_ff48_4da6_90c2_a63721a78753  Operator=square  SaturateOnIntegerOverflow=on
  Math Function1 : Math  RequirementInfo={} %GIDa_b9819a57_c6fa_43b1_ab91_7ea628f70e8b  Operator=square  SaturateOnIntegerOverflow=on
  Merge : Merge
  Relational Operator : RelationalOperator  RequirementInfo={} %GIDa_27550b50_4055_429e_b5b7_5e14144443ec  Operator=<  OutDataTypeStr=boolean
  Relational Operator1 : RelationalOperator  RequirementInfo={} %GIDa_7711719a_10c4_45df_a871_962bc5b69dee  Operator=>  OutDataTypeStr=boolean
  RollCnt_Qulfr_Calc : Subsystem  RequirementInfo={'linktype_rmi_doors' '0000cf65 (/E-STEER Core/SubSystem Specifications/Electrical Actuator/Control Module/FDD Module Requirements/EA4/ES241A_MotAg2Meas)' '#ES241A_137' 'true' 'REQ: ES241A_137' '' } %GIDa_33ff3977_32e1_4c6a_9b10_7c1eae4bf9d3
  Subtract : Sum  RequirementInfo={} %GIDa_5276e5a2_38e4_4ed2_9556_3a5cec1d82d4  Inputs=+-
  Subtract1 : Sum  RequirementInfo={} %GIDa_e3d875ef_18cb_48f8_9516_b746105cb350  Inputs=+-
  TestFail : Subsystem  TreatAsAtomicUnit=on
  TestPass : Subsystem  RequirementInfo={'linktype_rmi_doors' '0000cf65 (/E-STEER Core/SubSystem Specifications/Electrical Actuator/Control Module/FDD Module Requirements/EA4/ES241A_MotAg2Meas)' '#ES241A_134' 'true' 'REQ: ES241A_134' '' } %GIDa_271733fb_38d3_4643_afe9_1452c2b57714  TreatAsAtomicUnit=on
  MotAg2MeclQlfr : Outport
  MotAg2MeclRollgCntr : Outport  Port=2
  MotPosTestOk_Cnt : Outport  Port=3
  MotAg2VltgSqd : Outport  Port=4
  wires:
  Math Function/1 -> Add/1
  MotAg2Sin/1 -> Subtract/1
  Math Function1/1 -> Add/2
  Subtract/1 -> Math Function/1
  MotAg2Cos/1 -> Subtract1/1
  Subtract1/1 -> Math Function1/1
  Relational Operator1/1 -> [MotAg2MaxThdTrue], Logical Operator/2
  Relational Operator/1 -> [MotAg2MinThdTrue], Logical Operator/1
  [MotAg2MinThdTrue] -> TestFail/1(SinCosMinErr)
  [MotAg2MaxThdTrue] -> TestFail/2(SinCosMaxErr)
  If/1 -> TestFail/Action
  If/2 -> TestPass/Action
  RollCnt_Qulfr_Calc/1(MotAg2MeclQlfr) -> MotAg2MeclQlfr/1
  RollCnt_Qulfr_Calc/2(MotAg2MeclRollgCntr) -> MotAg2MeclRollgCntr/1
  TestFail/1(FailParamByte) -> Merge/1
  TestPass/1(PassParamByte) -> Merge/2
  Merge/1 -> RollCnt_Qulfr_Calc/1(ParamByte)
  Logical Operator/1 -> Logical Operator1/1, If/1
  Constant/1 -> Relational Operator/2
  Constant1/1 -> Relational Operator1/2
  MotAg2CosAdcFaild/1 -> [CosAdcFaild], Logical Operator/4
  Logical Operator1/1 -> MotPosTestOk_Cnt/1
  MotAg2SinAdcFaild/1 -> [SinAdcFaild], Logical Operator/3
  [SinAdcFaild] -> TestFail/3(SinAdcFaild)
  [CosAdcFaild] -> TestFail/4(CosAdcFaild)
  Add/1 -> Relational Operator1/1, LimStat_f1/1, Relational Operator/1
  LimStat_f1/1 -> MotAg2VltgSqd/1
  Data Store Read/1 -> Subtract/2
  Data Store Read1/1 -> Subtract1/2

== system ES241A_MotAg2Meas/MotAg2Meas/MotAg2MeasPer1/CopyRight2 ==

== system ES241A_MotAg2Meas/MotAg2Meas/MotAg2MeasPer1/FltInj_f32 ==
  note: This block requires no modification by FDD author.
      |
      | This block does not actually simulate any fault injection.  It is simply a pass-thru.
      |
      | The Constant port (#2) simply terminates its signal, but we are trying to force the FDD author
      | to properly use the FltInjectionLocType enumeration in FDD model.
  note: EA4.x Fault Injection
  Signal_In : Inport
  Constant : Inport  Port=2
  CopyRight2 : Subsystem  Description=|  mask(Copyright Information){none=on}
      | Copyright info block.                                               
      |                                                                     
      | Place copyright information at the top of every subsystem in design.
      mask prompts: none "No parameters"
      mask help: Place copyright information at the top of every subsystem in design.
      mask Display:
      | NxtrConf = 'Nexteer Confidential';
      | 
      | sys = bdroot; %handle for the current model ("system")
      | first = get_param(sys,'Created');
      | first = first(end-3:end);  %year is last four digits
      | 
      | last = get_param(sys,'LastModifiedDate');
      | if isempty(last)
      |     last = datestr(now,'yyyy');
      | else
      |     last = last(end-3:end);
      | end
      | 
      | if strcmp(first,last)
      |     fprintf('%s -- Copyright %s Nexteer',NxtrConf,first)
      | else
      |     fprintf('%s -- %s%s- %s Nexteer',NxtrConf,char(169),first,last)
      | end
  Terminator : Terminator
  Signal_Out : Outport
  wires:
  Signal_In/1 -> Signal_Out/1
  Constant/1 -> Terminator/1

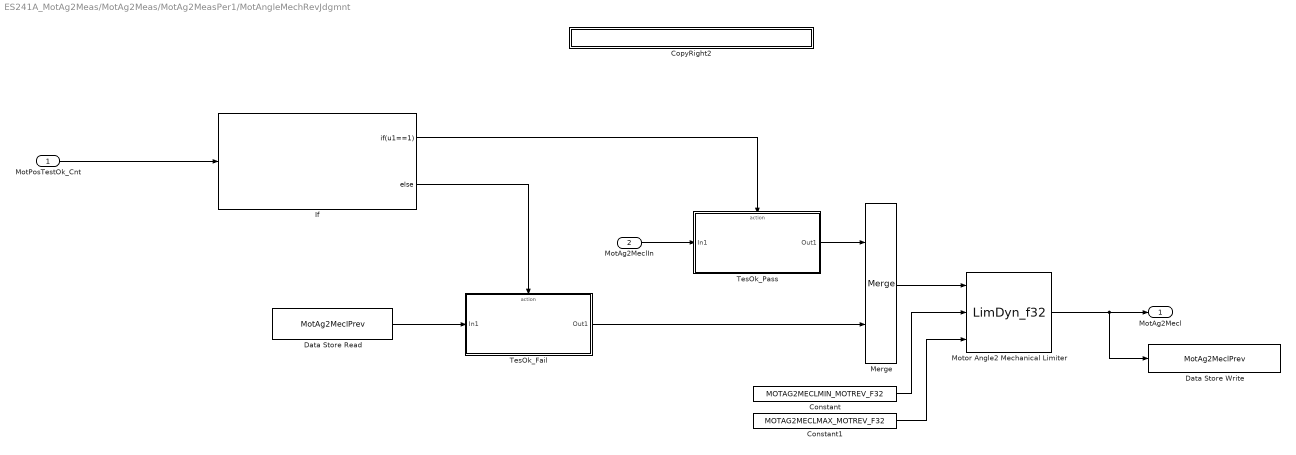
== system ES241A_MotAg2Meas/MotAg2Meas/MotAg2MeasPer1/MotAngleMechRevJdgmnt ==
  MotPosTestOk_Cnt : Inport
  MotAg2MeclIn : Inport  Port=2
  Constant : Constant  Value=MOTAG2MECLMIN_MOTREV_F32
  Constant1 : Constant  Value=MOTAG2MECLMAX_MOTREV_F32
  CopyRight2 : Subsystem  Description=|  mask(Copyright Information){none=on}
      | Copyright info block.                                               
      |                                                                     
      | Place copyright information at the top of every subsystem in design.
      mask prompts: none "No parameters"
      mask help: Place copyright information at the top of every subsystem in design.
      mask Display:
      | NxtrConf = 'Nexteer Confidential';
      | 
      | sys = bdroot; %handle for the current model ("system")
      | first = get_param(sys,'Created');
      | if(isempty(first))
      |     first = datestr(now,'yyyy');
      | else
      |     first = first(end-3:end);  %year is last four digits
      | end
      | 
      | last = get_param(sys,'LastModifiedDate');
      | if isempty(last)
      |     last = datestr(now,'yyyy');
      | else
      |     last = last(end-3:end);
      | end
      | 
      | if strcmp(first,last)
      |     fprintf('%s -- Copyright %s Nexteer',NxtrConf,first)
      | else
      |     fprintf('%s -- %s%s- %s Nexteer',NxtrConf,char(169),first,last)
      | end
  Data Store Read : DataStoreRead  DataStoreName=MotAg2MeclPrev
  Data Store Write : DataStoreWrite  DataStoreName=MotAg2MeclPrev
  If : If  IfExpression=u1==1
  Merge : Merge
  Motor Angle2 Mechanical Limiter : NxtrLim/LimDyn_f32  RequirementInfo={} %GIDa_75ae07f5_a2cf_4ea5_8b98_ca00063f41df
  TesOk_Fail : Subsystem  RequirementInfo={'linktype_rmi_doors' '0000cf65 (/E-STEER Core/SubSystem Specifications/Electrical Actuator/Control Module/FDD Module Requirements/EA4/ES241A_MotAg2Meas)' '#ES241A_147' 'true' 'REQ: ES241A_147' '' ; 'linktype_rmi_doors' '0000cf65 (/E-STEER Core/SubSystem Specifications/Electrical Actuator/Control Module/FDD Module Requirements/EA4/ES241A_MotAg2Meas)' '#ES241A_148' 'true' 'REQ: ES241A_148' '' ; 'linktype_rmi_doors' '0000cf65 (/E-STEER Core/SubSystem Specifications/Electrical Actuator/Control Module/FDD Module Requirements/EA4/ES241A_MotAg2Meas)' '#ES241A_139' 'true' 'REQ: ES241A_139' '' } %GIDa_0f0b4bd1_cd3b_42b9_a419_c238b2e3f366  TreatAsAtomicUnit=on
  TesOk_Pass : Subsystem  TreatAsAtomicUnit=on
  MotAg2Mecl : Outport
  wires:
  If/1 -> TesOk_Pass/Action
  If/2 -> TesOk_Fail/Action
  TesOk_Pass/1(Out1) -> Merge/1
  TesOk_Fail/1(Out1) -> Merge/2
  Data Store Read/1 -> TesOk_Fail/1(In1)
  MotPosTestOk_Cnt/1 -> If/1
  MotAg2MeclIn/1 -> TesOk_Pass/1(In1)
  Merge/1 -> Motor Angle2 Mechanical Limiter/1
  Motor Angle2 Mechanical Limiter/1 -> Data Store Write/1, MotAg2Mecl/1
  Constant/1 -> Motor Angle2 Mechanical Limiter/2
  Constant1/1 -> Motor Angle2 Mechanical Limiter/3

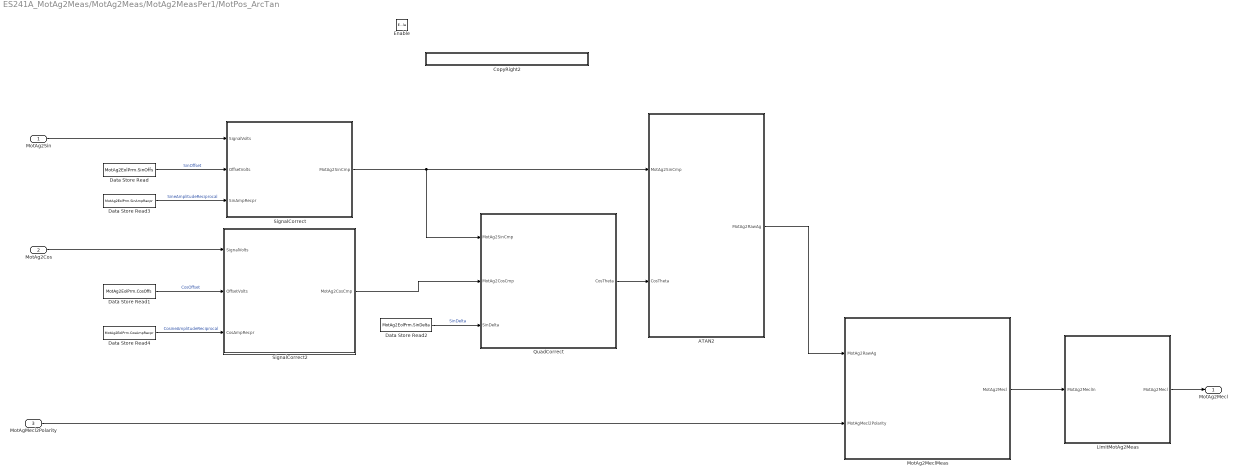
== system ES241A_MotAg2Meas/MotAg2Meas/MotAg2MeasPer1/MotPos_ArcTan ==
  MotAg2Sin : Inport
  MotAg2Cos : Inport  Port=2
  MotAgMecl2Polarity : Inport  RequirementInfo={} %GIDa_f88c60fe_1722_4e27_ab61_8a7da6a73543  Port=3
  Enable : EnablePort
  ATAN2 : Subsystem  RequirementInfo={'linktype_rmi_doors' '0000cf65 (/E-STEER Core/SubSystem Specifications/Electrical Actuator/Control Module/FDD Module Requirements/EA4/ES241A_MotAg2Meas)' '#ES241A_123' 'true' 'REQ: ES241A_123' '' } %GIDa_4a37e0cf_c570_47cf_a8a6_a1060e3c63ea  TreatAsAtomicUnit=on
  CopyRight2 : Subsystem  Description=|  mask(Copyright Information){none=on}
      | Copyright info block.                                               
      |                                                                     
      | Place copyright information at the top of every subsystem in design.
      mask prompts: none "No parameters"
      mask help: Place copyright information at the top of every subsystem in design.
      mask Display:
      | NxtrConf = 'Nexteer Confidential';
      | 
      | sys = bdroot; %handle for the current model ("system")
      | first = get_param(sys,'Created');
      | if(isempty(first))
      |     first = datestr(now,'yyyy');
      | else
      |     first = first(end-3:end);  %year is last four digits
      | end
      | 
      | last = get_param(sys,'LastModifiedDate');
      | if isempty(last)
      |     last = datestr(now,'yyyy');
      | else
      |     last = last(end-3:end);
      | end
      | 
      | if strcmp(first,last)
      |     fprintf('%s -- Copyright %s Nexteer',NxtrConf,first)
      | else
      |     fprintf('%s -- %s%s- %s Nexteer',NxtrConf,char(169),first,last)
      | end
  Data Store Read : DataStoreRead  DataStoreName=MotAg2EolPrm  DataStoreElements=MotAg2EolPrm.SinOffs
  Data Store Read1 : DataStoreRead  DataStoreName=MotAg2EolPrm  DataStoreElements=MotAg2EolPrm.CosOffs
  Data Store Read2 : DataStoreRead  DataStoreName=MotAg2EolPrm  DataStoreElements=MotAg2EolPrm.SinDelta
  Data Store Read3 : DataStoreRead  DataStoreName=MotAg2EolPrm  DataStoreElements=MotAg2EolPrm.SinAmpRecpr
  Data Store Read4 : DataStoreRead  DataStoreName=MotAg2EolPrm  DataStoreElements=MotAg2EolPrm.CosAmpRecpr
  LimitMotAg2Meas : Subsystem
  MotAg2MeclMeas : Subsystem  RequirementInfo="{}  %GIDa_155eb0a8_c2ed_490a_af1d_f8f4e19f97e7"  TreatAsAtomicUnit=on
  QuadCorrect : Subsystem  RequirementInfo={'linktype_rmi_doors' '0000cf65 (/E-STEER Core/SubSystem Specifications/Electrical Actuator/Control Module/FDD Module Requirements/EA4/ES241A_MotAg2Meas)' '#ES241A_121' 'true' 'REQ: ES241A_121' '' } %GIDa_3d78f2b2_5c94_409f_934c_8aefaaebd76d  TreatAsAtomicUnit=on
  SignalCorrect : Subsystem  RequirementInfo={'linktype_rmi_doors' '0000cf65 (/E-STEER Core/SubSystem Specifications/Electrical Actuator/Control Module/FDD Module Requirements/EA4/ES241A_MotAg2Meas)' '#ES241A_117' 'true' 'REQ: ES241A_117' '' } %GIDa_8d0c5619_ebe6_40e3_89d6_85a8ef0fbaf9
  SignalCorrect2 : Subsystem  RequirementInfo={'linktype_rmi_doors' '0000cf65 (/E-STEER Core/SubSystem Specifications/Electrical Actuator/Control Module/FDD Module Requirements/EA4/ES241A_MotAg2Meas)' '#ES241A_83' 'true' 'REQ: ES241A_83' '' } %GIDa_07f3fc20_adc4_4d19_a2a9_4772ed53a785
  MotAg2Mecl : Outport  RequirementInfo="{}  %GIDa_dd9bd2af_a5c1_4575_89a6_d173bd83c2f9"
  wires:
  SignalCorrect/1(MotAg2SinCmp) -> QuadCorrect/1(MotAg2SinCmp), ATAN2/1(MotAg2SinCmp)
  ATAN2/1(MotAg2RawAg) -> MotAg2MeclMeas/1(MotAg2RawAg)
  MotAg2Cos/1 -> SignalCorrect2/1(SignalVolts)
  MotAgMecl2Polarity/1 -> MotAg2MeclMeas/2(MotAgMecl2Polarity)
  SignalCorrect2/1(MotAg2CosCmp) -> QuadCorrect/2(MotAg2CosCmp)
  Data Store Read/1 -> SignalCorrect/2(OffsetVolts)  "SinOffset"
  Data Store Read3/1 -> SignalCorrect/3(SinAmpRecpr)  "SineAmplitudeReciprocal"
  Data Store Read1/1 -> SignalCorrect2/2(OffsetVolts)  "CosOffset"
  Data Store Read4/1 -> SignalCorrect2/3(CosAmpRecpr)  "CosineAmplitudeReciprocal"
  Data Store Read2/1 -> QuadCorrect/3(SinDelta)  "SinDelta"
  MotAg2Sin/1 -> SignalCorrect/1(SignalVolts)
  MotAg2MeclMeas/1(MotAg2Mecl) -> LimitMotAg2Meas/1(MotAg2MeclIn)
  LimitMotAg2Meas/1(MotAg2Mecl) -> MotAg2Mecl/1
  QuadCorrect/1(CosTheta) -> ATAN2/2(CosTheta)

== system ES241A_MotAg2Meas/MotAg2Meas/MotAg2MeasInit1/MotAg2EolPrm_GetErrorStatus/CopyRight2 ==

== system ES241A_MotAg2Meas/MotAg2Meas/MotAg2MeasInit1/NVM_NOK/CopyRight2 ==

== system ES241A_MotAg2Meas/MotAg2Meas/MotAg2MeasInit1/NVM_Ok/CopyRight2 ==

== system ES241A_MotAg2Meas/MotAg2Meas/MotAg2MeasPer1/AnalogMsbDiagnostics/CopyRight2 ==
